simulink model "RADTRANS002"  (R2020b)
settings: Solver=VariableStepAuto  StartTime=0.0  StopTime=10.0  RelTol=1e-3
undefined symbols (not defined in the file): Line_110_C, Line_110_L, Line_110_R, Line_220_C, Line_220_L, Line_220_R, Line_35_C, Line_35_L, Line_35_R, Line_6_L, Line_6_R, Sys_f_Hz, Sys_V_net_kV, Tr_110_35_L_pu, Tr_110_35_R_pu, Tr_110_35_Sn_VA, Tr_110_35_V_HV_kV, Tr_110_35_V_LV_kV, Tr_110_6_L_pu, Tr_110_6_R_pu, Tr_110_6_Sn_VA, Tr_110_6_V_HV_kV, Tr_110_6_V_LV_kV, Tr_220_110_L_pu, Tr_220_110_R_pu, Tr_220_110_Sn_VA, Tr_220_110_V_HV_kV, Tr_220_110_V_LV_kV, Tr_35_04_L_pu, Tr_35_04_R_pu, Tr_35_04_Sn_VA, Tr_35_04_V_HV_kV, Tr_35_04_V_LV_kV, Tr_6_04_L_pu, Tr_6_04_R_pu, Tr_6_04_Sn_VA, Tr_6_04_V_HV_kV, Tr_6_04_V_LV_kV, Ts_powergui
libraries: dspstat3 x288, powerlib x202, powerlib_meascontrol x72
(part 1 of 7)
settings Model: Creator=New-life  LastModifiedBy=New-life

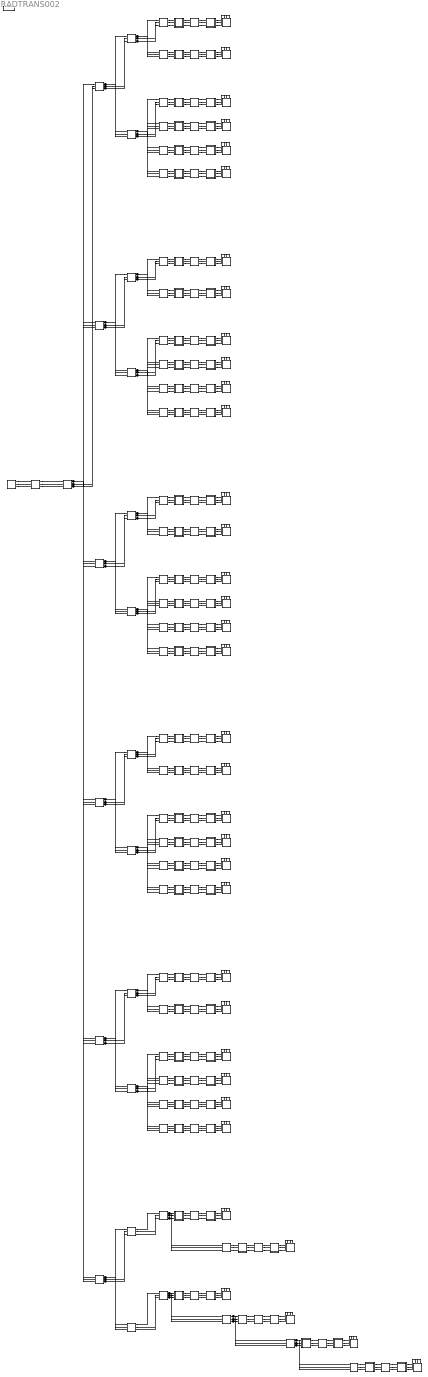
== system RADTRANS002 ==
  M_IN_Город_1_1 : Subsystem
      settings: CopyFcn=|
      | % Получаем путь и имя нового (только что скопированного) блока
      | blockPath = gcb;
      | blockName = get_param(blockPath, 'Name');
      | 
      | % Ищем число в названии самой подсистемы (например, берем "2" из "Measure_2")
      | numStr = regexp(blockName, '\d+', 'match');
      | 
      | if ~isempty(numStr)
      |     newNum = numStr{end}; % Берем последнее найденное число
      | 
      |     % --- 1. Обновляем скрытые теги в Goto и From (радиочастоты) ---
      |     gotos = find_system(blockPath, 'LookUnderMasks', 'on', 'BlockType', 'Goto');
      |     froms = find_system(blockPath, 'LookUnderMasks', 'on', 'BlockType', 'From');
      | 
      |     for i = 1:length(gotos)
      |         oldTag = get_param(gotos{i}, 'GotoTag');
      |         set_param(gotos{i}, 'GotoTag', regexprep(oldTag, '\d+$', newNum));
      |     end
      |     for i = 1:length(froms)
      |         oldTag = get_param(froms{i}, 'GotoTag');
      |         set_param(froms{i}, 'GotoTag', regexprep(oldTag, '\d+$', newNum));
      |     end
      | 
      |     % --- 2. ПЕРЕИМЕНОВЫВАЕМ САМИ БЛОКИ (визуальные надписи UI0 -> UI1 и т.д.) ---
      |     % Ищем все элементы только внутри этой подсистемы
      |     internalBlocks = find_system(blockPath, 'SearchDepth', 1, 'LookUnderMasks', 'on');
      | 
      |     % Цикл начинаем с 2, так как 1-й элемент в списке - это сама папка подсистемы
      |     for i = 2:length(internalBlocks)
      |         oldName = get_param(internalBlocks{i}, 'Name');
      |         % Ищем цифру в конце имени и меняем на новую
      |         newName = regexprep(oldName, '\d+$', newNum);
      | 
      |         % Если имя изменилось, применяем его
      |         if ~strcmp(oldName, newName)
      |             try
      |                 set_param(internalBlocks{i}, 'Name', newName);
      |             catch
      |                 % Игнорируем ошибку, если вдруг такое имя уже случайно есть
      |             end
      |         end
      |     end
      | end
  M_IN_Город_1_2 : Subsystem
      settings: CopyFcn=|
      | % Получаем путь и имя нового (только что скопированного) блока
      | blockPath = gcb;
      | blockName = get_param(blockPath, 'Name');
      | 
      | % Ищем число в названии самой подсистемы (например, берем "2" из "Measure_2")
      | numStr = regexp(blockName, '\d+', 'match');
      | 
      | if ~isempty(numStr)
      |     newNum = numStr{end}; % Берем последнее найденное число
      | 
      |     % --- 1. Обновляем скрытые теги в Goto и From (радиочастоты) ---
      |     gotos = find_system(blockPath, 'LookUnderMasks', 'on', 'BlockType', 'Goto');
      |     froms = find_system(blockPath, 'LookUnderMasks', 'on', 'BlockType', 'From');
      | 
      |     for i = 1:length(gotos)
      |         oldTag = get_param(gotos{i}, 'GotoTag');
      |         set_param(gotos{i}, 'GotoTag', regexprep(oldTag, '\d+$', newNum));
      |     end
      |     for i = 1:length(froms)
      |         oldTag = get_param(froms{i}, 'GotoTag');
      |         set_param(froms{i}, 'GotoTag', regexprep(oldTag, '\d+$', newNum));
      |     end
      | 
      |     % --- 2. ПЕРЕИМЕНОВЫВАЕМ САМИ БЛОКИ (визуальные надписи UI0 -> UI1 и т.д.) ---
      |     % Ищем все элементы только внутри этой подсистемы
      |     internalBlocks = find_system(blockPath, 'SearchDepth', 1, 'LookUnderMasks', 'on');
      | 
      |     % Цикл начинаем с 2, так как 1-й элемент в списке - это сама папка подсистемы
      |     for i = 2:length(internalBlocks)
      |         oldName = get_param(internalBlocks{i}, 'Name');
      |         % Ищем цифру в конце имени и меняем на новую
      |         newName = regexprep(oldName, '\d+$', newNum);
      | 
      |         % Если имя изменилось, применяем его
      |         if ~strcmp(oldName, newName)
      |             try
      |                 set_param(internalBlocks{i}, 'Name', newName);
      |             catch
      |                 % Игнорируем ошибку, если вдруг такое имя уже случайно есть
      |             end
      |         end
      |     end
      | end
  M_IN_Город_1_3 : Subsystem
      settings: CopyFcn=|
      | % Получаем путь и имя нового (только что скопированного) блока
      | blockPath = gcb;
      | blockName = get_param(blockPath, 'Name');
      | 
      | % Ищем число в названии самой подсистемы (например, берем "2" из "Measure_2")
      | numStr = regexp(blockName, '\d+', 'match');
      | 
      | if ~isempty(numStr)
      |     newNum = numStr{end}; % Берем последнее найденное число
      | 
      |     % --- 1. Обновляем скрытые теги в Goto и From (радиочастоты) ---
      |     gotos = find_system(blockPath, 'LookUnderMasks', 'on', 'BlockType', 'Goto');
      |     froms = find_system(blockPath, 'LookUnderMasks', 'on', 'BlockType', 'From');
      | 
      |     for i = 1:length(gotos)
      |         oldTag = get_param(gotos{i}, 'GotoTag');
      |         set_param(gotos{i}, 'GotoTag', regexprep(oldTag, '\d+$', newNum));
      |     end
      |     for i = 1:length(froms)
      |         oldTag = get_param(froms{i}, 'GotoTag');
      |         set_param(froms{i}, 'GotoTag', regexprep(oldTag, '\d+$', newNum));
      |     end
      | 
      |     % --- 2. ПЕРЕИМЕНОВЫВАЕМ САМИ БЛОКИ (визуальные надписи UI0 -> UI1 и т.д.) ---
      |     % Ищем все элементы только внутри этой подсистемы
      |     internalBlocks = find_system(blockPath, 'SearchDepth', 1, 'LookUnderMasks', 'on');
      | 
      |     % Цикл начинаем с 2, так как 1-й элемент в списке - это сама папка подсистемы
      |     for i = 2:length(internalBlocks)
      |         oldName = get_param(internalBlocks{i}, 'Name');
      |         % Ищем цифру в конце имени и меняем на новую
      |         newName = regexprep(oldName, '\d+$', newNum);
      | 
      |         % Если имя изменилось, применяем его
      |         if ~strcmp(oldName, newName)
      |             try
      |                 set_param(internalBlocks{i}, 'Name', newName);
      |             catch
      |                 % Игнорируем ошибку, если вдруг такое имя уже случайно есть
      |             end
      |         end
      |     end
      | end
  M_IN_Город_1_4 : Subsystem
      settings: CopyFcn=|
      | % Получаем путь и имя нового (только что скопированного) блока
      | blockPath = gcb;
      | blockName = get_param(blockPath, 'Name');
      | 
      | % Ищем число в названии самой подсистемы (например, берем "2" из "Measure_2")
      | numStr = regexp(blockName, '\d+', 'match');
      | 
      | if ~isempty(numStr)
      |     newNum = numStr{end}; % Берем последнее найденное число
      | 
      |     % --- 1. Обновляем скрытые теги в Goto и From (радиочастоты) ---
      |     gotos = find_system(blockPath, 'LookUnderMasks', 'on', 'BlockType', 'Goto');
      |     froms = find_system(blockPath, 'LookUnderMasks', 'on', 'BlockType', 'From');
      | 
      |     for i = 1:length(gotos)
      |         oldTag = get_param(gotos{i}, 'GotoTag');
      |         set_param(gotos{i}, 'GotoTag', regexprep(oldTag, '\d+$', newNum));
      |     end
      |     for i = 1:length(froms)
      |         oldTag = get_param(froms{i}, 'GotoTag');
      |         set_param(froms{i}, 'GotoTag', regexprep(oldTag, '\d+$', newNum));
      |     end
      | 
      |     % --- 2. ПЕРЕИМЕНОВЫВАЕМ САМИ БЛОКИ (визуальные надписи UI0 -> UI1 и т.д.) ---
      |     % Ищем все элементы только внутри этой подсистемы
      |     internalBlocks = find_system(blockPath, 'SearchDepth', 1, 'LookUnderMasks', 'on');
      | 
      |     % Цикл начинаем с 2, так как 1-й элемент в списке - это сама папка подсистемы
      |     for i = 2:length(internalBlocks)
      |         oldName = get_param(internalBlocks{i}, 'Name');
      |         % Ищем цифру в конце имени и меняем на новую
      |         newName = regexprep(oldName, '\d+$', newNum);
      | 
      |         % Если имя изменилось, применяем его
      |         if ~strcmp(oldName, newName)
      |             try
      |                 set_param(internalBlocks{i}, 'Name', newName);
      |             catch
      |                 % Игнорируем ошибку, если вдруг такое имя уже случайно есть
      |             end
      |         end
      |     end
      | end
  M_IN_Город_2_1 : Subsystem
      settings: CopyFcn=|
      | % Получаем путь и имя нового (только что скопированного) блока
      | blockPath = gcb;
      | blockName = get_param(blockPath, 'Name');
      | 
      | % Ищем число в названии самой подсистемы (например, берем "2" из "Measure_2")
      | numStr = regexp(blockName, '\d+', 'match');
      | 
      | if ~isempty(numStr)
      |     newNum = numStr{end}; % Берем последнее найденное число
      | 
      |     % --- 1. Обновляем скрытые теги в Goto и From (радиочастоты) ---
      |     gotos = find_system(blockPath, 'LookUnderMasks', 'on', 'BlockType', 'Goto');
      |     froms = find_system(blockPath, 'LookUnderMasks', 'on', 'BlockType', 'From');
      | 
      |     for i = 1:length(gotos)
      |         oldTag = get_param(gotos{i}, 'GotoTag');
      |         set_param(gotos{i}, 'GotoTag', regexprep(oldTag, '\d+$', newNum));
      |     end
      |     for i = 1:length(froms)
      |         oldTag = get_param(froms{i}, 'GotoTag');
      |         set_param(froms{i}, 'GotoTag', regexprep(oldTag, '\d+$', newNum));
      |     end
      | 
      |     % --- 2. ПЕРЕИМЕНОВЫВАЕМ САМИ БЛОКИ (визуальные надписи UI0 -> UI1 и т.д.) ---
      |     % Ищем все элементы только внутри этой подсистемы
      |     internalBlocks = find_system(blockPath, 'SearchDepth', 1, 'LookUnderMasks', 'on');
      | 
      |     % Цикл начинаем с 2, так как 1-й элемент в списке - это сама папка подсистемы
      |     for i = 2:length(internalBlocks)
      |         oldName = get_param(internalBlocks{i}, 'Name');
      |         % Ищем цифру в конце имени и меняем на новую
      |         newName = regexprep(oldName, '\d+$', newNum);
      | 
      |         % Если имя изменилось, применяем его
      |         if ~strcmp(oldName, newName)
      |             try
      |                 set_param(internalBlocks{i}, 'Name', newName);
      |             catch
      |                 % Игнорируем ошибку, если вдруг такое имя уже случайно есть
      |             end
      |         end
      |     end
      | end
  M_IN_Город_2_2 : Subsystem
      settings: CopyFcn=|
      | % Получаем путь и имя нового (только что скопированного) блока
      | blockPath = gcb;
      | blockName = get_param(blockPath, 'Name');
      | 
      | % Ищем число в названии самой подсистемы (например, берем "2" из "Measure_2")
      | numStr = regexp(blockName, '\d+', 'match');
      | 
      | if ~isempty(numStr)
      |     newNum = numStr{end}; % Берем последнее найденное число
      | 
      |     % --- 1. Обновляем скрытые теги в Goto и From (радиочастоты) ---
      |     gotos = find_system(blockPath, 'LookUnderMasks', 'on', 'BlockType', 'Goto');
      |     froms = find_system(blockPath, 'LookUnderMasks', 'on', 'BlockType', 'From');
      | 
      |     for i = 1:length(gotos)
      |         oldTag = get_param(gotos{i}, 'GotoTag');
      |         set_param(gotos{i}, 'GotoTag', regexprep(oldTag, '\d+$', newNum));
      |     end
      |     for i = 1:length(froms)
      |         oldTag = get_param(froms{i}, 'GotoTag');
      |         set_param(froms{i}, 'GotoTag', regexprep(oldTag, '\d+$', newNum));
      |     end
      | 
      |     % --- 2. ПЕРЕИМЕНОВЫВАЕМ САМИ БЛОКИ (визуальные надписи UI0 -> UI1 и т.д.) ---
      |     % Ищем все элементы только внутри этой подсистемы
      |     internalBlocks = find_system(blockPath, 'SearchDepth', 1, 'LookUnderMasks', 'on');
      | 
      |     % Цикл начинаем с 2, так как 1-й элемент в списке - это сама папка подсистемы
      |     for i = 2:length(internalBlocks)
      |         oldName = get_param(internalBlocks{i}, 'Name');
      |         % Ищем цифру в конце имени и меняем на новую
      |         newName = regexprep(oldName, '\d+$', newNum);
      | 
      |         % Если имя изменилось, применяем его
      |         if ~strcmp(oldName, newName)
      |             try
      |                 set_param(internalBlocks{i}, 'Name', newName);
      |             catch
      |                 % Игнорируем ошибку, если вдруг такое имя уже случайно есть
      |             end
      |         end
      |     end
      | end
  M_IN_Город_2_3 : Subsystem
      settings: CopyFcn=|
      | % Получаем путь и имя нового (только что скопированного) блока
      | blockPath = gcb;
      | blockName = get_param(blockPath, 'Name');
      | 
      | % Ищем число в названии самой подсистемы (например, берем "2" из "Measure_2")
      | numStr = regexp(blockName, '\d+', 'match');
      | 
      | if ~isempty(numStr)
      |     newNum = numStr{end}; % Берем последнее найденное число
      | 
      |     % --- 1. Обновляем скрытые теги в Goto и From (радиочастоты) ---
      |     gotos = find_system(blockPath, 'LookUnderMasks', 'on', 'BlockType', 'Goto');
      |     froms = find_system(blockPath, 'LookUnderMasks', 'on', 'BlockType', 'From');
      | 
      |     for i = 1:length(gotos)
      |         oldTag = get_param(gotos{i}, 'GotoTag');
      |         set_param(gotos{i}, 'GotoTag', regexprep(oldTag, '\d+$', newNum));
      |     end
      |     for i = 1:length(froms)
      |         oldTag = get_param(froms{i}, 'GotoTag');
      |         set_param(froms{i}, 'GotoTag', regexprep(oldTag, '\d+$', newNum));
      |     end
      | 
      |     % --- 2. ПЕРЕИМЕНОВЫВАЕМ САМИ БЛОКИ (визуальные надписи UI0 -> UI1 и т.д.) ---
      |     % Ищем все элементы только внутри этой подсистемы
      |     internalBlocks = find_system(blockPath, 'SearchDepth', 1, 'LookUnderMasks', 'on');
      | 
      |     % Цикл начинаем с 2, так как 1-й элемент в списке - это сама папка подсистемы
      |     for i = 2:length(internalBlocks)
      |         oldName = get_param(internalBlocks{i}, 'Name');
      |         % Ищем цифру в конце имени и меняем на новую
      |         newName = regexprep(oldName, '\d+$', newNum);
      | 
      |         % Если имя изменилось, применяем его
      |         if ~strcmp(oldName, newName)
      |             try
      |                 set_param(internalBlocks{i}, 'Name', newName);
      |             catch
      |                 % Игнорируем ошибку, если вдруг такое имя уже случайно есть
      |             end
      |         end
      |     end
      | end
  M_IN_Город_2_4 : Subsystem
      settings: CopyFcn=|
      | % Получаем путь и имя нового (только что скопированного) блока
      | blockPath = gcb;
      | blockName = get_param(blockPath, 'Name');
      | 
      | % Ищем число в названии самой подсистемы (например, берем "2" из "Measure_2")
      | numStr = regexp(blockName, '\d+', 'match');
      | 
      | if ~isempty(numStr)
      |     newNum = numStr{end}; % Берем последнее найденное число
      | 
      |     % --- 1. Обновляем скрытые теги в Goto и From (радиочастоты) ---
      |     gotos = find_system(blockPath, 'LookUnderMasks', 'on', 'BlockType', 'Goto');
      |     froms = find_system(blockPath, 'LookUnderMasks', 'on', 'BlockType', 'From');
      | 
      |     for i = 1:length(gotos)
      |         oldTag = get_param(gotos{i}, 'GotoTag');
      |         set_param(gotos{i}, 'GotoTag', regexprep(oldTag, '\d+$', newNum));
      |     end
      |     for i = 1:length(froms)
      |         oldTag = get_param(froms{i}, 'GotoTag');
      |         set_param(froms{i}, 'GotoTag', regexprep(oldTag, '\d+$', newNum));
      |     end
      | 
      |     % --- 2. ПЕРЕИМЕНОВЫВАЕМ САМИ БЛОКИ (визуальные надписи UI0 -> UI1 и т.д.) ---
      |     % Ищем все элементы только внутри этой подсистемы
      |     internalBlocks = find_system(blockPath, 'SearchDepth', 1, 'LookUnderMasks', 'on');
      | 
      |     % Цикл начинаем с 2, так как 1-й элемент в списке - это сама папка подсистемы
      |     for i = 2:length(internalBlocks)
      |         oldName = get_param(internalBlocks{i}, 'Name');
      |         % Ищем цифру в конце имени и меняем на новую
      |         newName = regexprep(oldName, '\d+$', newNum);
      | 
      |         % Если имя изменилось, применяем его
      |         if ~strcmp(oldName, newName)
      |             try
      |                 set_param(internalBlocks{i}, 'Name', newName);
      |             catch
      |                 % Игнорируем ошибку, если вдруг такое имя уже случайно есть
      |             end
      |         end
      |     end
      | end
  M_IN_Город_3_1 : Subsystem
      settings: CopyFcn=|
      | % Получаем путь и имя нового (только что скопированного) блока
      | blockPath = gcb;
      | blockName = get_param(blockPath, 'Name');
      | 
      | % Ищем число в названии самой подсистемы (например, берем "2" из "Measure_2")
      | numStr = regexp(blockName, '\d+', 'match');
      | 
      | if ~isempty(numStr)
      |     newNum = numStr{end}; % Берем последнее найденное число
      | 
      |     % --- 1. Обновляем скрытые теги в Goto и From (радиочастоты) ---
      |     gotos = find_system(blockPath, 'LookUnderMasks', 'on', 'BlockType', 'Goto');
      |     froms = find_system(blockPath, 'LookUnderMasks', 'on', 'BlockType', 'From');
      | 
      |     for i = 1:length(gotos)
      |         oldTag = get_param(gotos{i}, 'GotoTag');
      |         set_param(gotos{i}, 'GotoTag', regexprep(oldTag, '\d+$', newNum));
      |     end
      |     for i = 1:length(froms)
      |         oldTag = get_param(froms{i}, 'GotoTag');
      |         set_param(froms{i}, 'GotoTag', regexprep(oldTag, '\d+$', newNum));
      |     end
      | 
      |     % --- 2. ПЕРЕИМЕНОВЫВАЕМ САМИ БЛОКИ (визуальные надписи UI0 -> UI1 и т.д.) ---
      |     % Ищем все элементы только внутри этой подсистемы
      |     internalBlocks = find_system(blockPath, 'SearchDepth', 1, 'LookUnderMasks', 'on');
      | 
      |     % Цикл начинаем с 2, так как 1-й элемент в списке - это сама папка подсистемы
      |     for i = 2:length(internalBlocks)
      |         oldName = get_param(internalBlocks{i}, 'Name');
      |         % Ищем цифру в конце имени и меняем на новую
      |         newName = regexprep(oldName, '\d+$', newNum);
      | 
      |         % Если имя изменилось, применяем его
      |         if ~strcmp(oldName, newName)
      |             try
      |                 set_param(internalBlocks{i}, 'Name', newName);
      |             catch
      |                 % Игнорируем ошибку, если вдруг такое имя уже случайно есть
      |             end
      |         end
      |     end
      | end
  M_IN_Город_3_2 : Subsystem
      settings: CopyFcn=|
      | % Получаем путь и имя нового (только что скопированного) блока
      | blockPath = gcb;
      | blockName = get_param(blockPath, 'Name');
      | 
      | % Ищем число в названии самой подсистемы (например, берем "2" из "Measure_2")
      | numStr = regexp(blockName, '\d+', 'match');
      | 
      | if ~isempty(numStr)
      |     newNum = numStr{end}; % Берем последнее найденное число
      | 
      |     % --- 1. Обновляем скрытые теги в Goto и From (радиочастоты) ---
      |     gotos = find_system(blockPath, 'LookUnderMasks', 'on', 'BlockType', 'Goto');
      |     froms = find_system(blockPath, 'LookUnderMasks', 'on', 'BlockType', 'From');
      | 
      |     for i = 1:length(gotos)
      |         oldTag = get_param(gotos{i}, 'GotoTag');
      |         set_param(gotos{i}, 'GotoTag', regexprep(oldTag, '\d+$', newNum));
      |     end
      |     for i = 1:length(froms)
      |         oldTag = get_param(froms{i}, 'GotoTag');
      |         set_param(froms{i}, 'GotoTag', regexprep(oldTag, '\d+$', newNum));
      |     end
      | 
      |     % --- 2. ПЕРЕИМЕНОВЫВАЕМ САМИ БЛОКИ (визуальные надписи UI0 -> UI1 и т.д.) ---
      |     % Ищем все элементы только внутри этой подсистемы
      |     internalBlocks = find_system(blockPath, 'SearchDepth', 1, 'LookUnderMasks', 'on');
      | 
      |     % Цикл начинаем с 2, так как 1-й элемент в списке - это сама папка подсистемы
      |     for i = 2:length(internalBlocks)
      |         oldName = get_param(internalBlocks{i}, 'Name');
      |         % Ищем цифру в конце имени и меняем на новую
      |         newName = regexprep(oldName, '\d+$', newNum);
      | 
      |         % Если имя изменилось, применяем его
      |         if ~strcmp(oldName, newName)
      |             try
      |                 set_param(internalBlocks{i}, 'Name', newName);
      |             catch
      |                 % Игнорируем ошибку, если вдруг такое имя уже случайно есть
      |             end
      |         end
      |     end
      | end
  M_IN_Город_3_3 : Subsystem
      settings: CopyFcn=|
      | % Получаем путь и имя нового (только что скопированного) блока
      | blockPath = gcb;
      | blockName = get_param(blockPath, 'Name');
      | 
      | % Ищем число в названии самой подсистемы (например, берем "2" из "Measure_2")
      | numStr = regexp(blockName, '\d+', 'match');
      | 
      | if ~isempty(numStr)
      |     newNum = numStr{end}; % Берем последнее найденное число
      | 
      |     % --- 1. Обновляем скрытые теги в Goto и From (радиочастоты) ---
      |     gotos = find_system(blockPath, 'LookUnderMasks', 'on', 'BlockType', 'Goto');
      |     froms = find_system(blockPath, 'LookUnderMasks', 'on', 'BlockType', 'From');
      | 
      |     for i = 1:length(gotos)
      |         oldTag = get_param(gotos{i}, 'GotoTag');
      |         set_param(gotos{i}, 'GotoTag', regexprep(oldTag, '\d+$', newNum));
      |     end
      |     for i = 1:length(froms)
      |         oldTag = get_param(froms{i}, 'GotoTag');
      |         set_param(froms{i}, 'GotoTag', regexprep(oldTag, '\d+$', newNum));
      |     end
      | 
      |     % --- 2. ПЕРЕИМЕНОВЫВАЕМ САМИ БЛОКИ (визуальные надписи UI0 -> UI1 и т.д.) ---
      |     % Ищем все элементы только внутри этой подсистемы
      |     internalBlocks = find_system(blockPath, 'SearchDepth', 1, 'LookUnderMasks', 'on');
      | 
      |     % Цикл начинаем с 2, так как 1-й элемент в списке - это сама папка подсистемы
      |     for i = 2:length(internalBlocks)
      |         oldName = get_param(internalBlocks{i}, 'Name');
      |         % Ищем цифру в конце имени и меняем на новую
      |         newName = regexprep(oldName, '\d+$', newNum);
      | 
      |         % Если имя изменилось, применяем его
      |         if ~strcmp(oldName, newName)
      |             try
      |                 set_param(internalBlocks{i}, 'Name', newName);
      |             catch
      |                 % Игнорируем ошибку, если вдруг такое имя уже случайно есть
      |             end
      |         end
      |     end
      | end
  M_IN_Город_3_4 : Subsystem
      settings: CopyFcn=|
      | % Получаем путь и имя нового (только что скопированного) блока
      | blockPath = gcb;
      | blockName = get_param(blockPath, 'Name');
      | 
      | % Ищем число в названии самой подсистемы (например, берем "2" из "Measure_2")
      | numStr = regexp(blockName, '\d+', 'match');
      | 
      | if ~isempty(numStr)
      |     newNum = numStr{end}; % Берем последнее найденное число
      | 
      |     % --- 1. Обновляем скрытые теги в Goto и From (радиочастоты) ---
      |     gotos = find_system(blockPath, 'LookUnderMasks', 'on', 'BlockType', 'Goto');
      |     froms = find_system(blockPath, 'LookUnderMasks', 'on', 'BlockType', 'From');
      | 
      |     for i = 1:length(gotos)
      |         oldTag = get_param(gotos{i}, 'GotoTag');
      |         set_param(gotos{i}, 'GotoTag', regexprep(oldTag, '\d+$', newNum));
      |     end
      |     for i = 1:length(froms)
      |         oldTag = get_param(froms{i}, 'GotoTag');
      |         set_param(froms{i}, 'GotoTag', regexprep(oldTag, '\d+$', newNum));
      |     end
      | 
      |     % --- 2. ПЕРЕИМЕНОВЫВАЕМ САМИ БЛОКИ (визуальные надписи UI0 -> UI1 и т.д.) ---
      |     % Ищем все элементы только внутри этой подсистемы
      |     internalBlocks = find_system(blockPath, 'SearchDepth', 1, 'LookUnderMasks', 'on');
      | 
      |     % Цикл начинаем с 2, так как 1-й элемент в списке - это сама папка подсистемы
      |     for i = 2:length(internalBlocks)
      |         oldName = get_param(internalBlocks{i}, 'Name');
      |         % Ищем цифру в конце имени и меняем на новую
      |         newName = regexprep(oldName, '\d+$', newNum);
      | 
      |         % Если имя изменилось, применяем его
      |         if ~strcmp(oldName, newName)
      |             try
      |                 set_param(internalBlocks{i}, 'Name', newName);
      |             catch
      |                 % Игнорируем ошибку, если вдруг такое имя уже случайно есть
      |             end
      |         end
      |     end
      | end
  M_IN_Город_4_1 : Subsystem
      settings: CopyFcn=|
      | % Получаем путь и имя нового (только что скопированного) блока
      | blockPath = gcb;
      | blockName = get_param(blockPath, 'Name');
      | 
      | % Ищем число в названии самой подсистемы (например, берем "2" из "Measure_2")
      | numStr = regexp(blockName, '\d+', 'match');
      | 
      | if ~isempty(numStr)
      |     newNum = numStr{end}; % Берем последнее найденное число
      | 
      |     % --- 1. Обновляем скрытые теги в Goto и From (радиочастоты) ---
      |     gotos = find_system(blockPath, 'LookUnderMasks', 'on', 'BlockType', 'Goto');
      |     froms = find_system(blockPath, 'LookUnderMasks', 'on', 'BlockType', 'From');
      | 
      |     for i = 1:length(gotos)
      |         oldTag = get_param(gotos{i}, 'GotoTag');
      |         set_param(gotos{i}, 'GotoTag', regexprep(oldTag, '\d+$', newNum));
      |     end
      |     for i = 1:length(froms)
      |         oldTag = get_param(froms{i}, 'GotoTag');
      |         set_param(froms{i}, 'GotoTag', regexprep(oldTag, '\d+$', newNum));
      |     end
      | 
      |     % --- 2. ПЕРЕИМЕНОВЫВАЕМ САМИ БЛОКИ (визуальные надписи UI0 -> UI1 и т.д.) ---
      |     % Ищем все элементы только внутри этой подсистемы
      |     internalBlocks = find_system(blockPath, 'SearchDepth', 1, 'LookUnderMasks', 'on');
      | 
      |     % Цикл начинаем с 2, так как 1-й элемент в списке - это сама папка подсистемы
      |     for i = 2:length(internalBlocks)
      |         oldName = get_param(internalBlocks{i}, 'Name');
      |         % Ищем цифру в конце имени и меняем на новую
      |         newName = regexprep(oldName, '\d+$', newNum);
      | 
      |         % Если имя изменилось, применяем его
      |         if ~strcmp(oldName, newName)
      |             try
      |                 set_param(internalBlocks{i}, 'Name', newName);
      |             catch
      |                 % Игнорируем ошибку, если вдруг такое имя уже случайно есть
      |             end
      |         end
      |     end
      | end
  M_IN_Город_4_2 : Subsystem
      settings: CopyFcn=|
      | % Получаем путь и имя нового (только что скопированного) блока
      | blockPath = gcb;
      | blockName = get_param(blockPath, 'Name');
      | 
      | % Ищем число в названии самой подсистемы (например, берем "2" из "Measure_2")
      | numStr = regexp(blockName, '\d+', 'match');
      | 
      | if ~isempty(numStr)
      |     newNum = numStr{end}; % Берем последнее найденное число
      | 
      |     % --- 1. Обновляем скрытые теги в Goto и From (радиочастоты) ---
      |     gotos = find_system(blockPath, 'LookUnderMasks', 'on', 'BlockType', 'Goto');
      |     froms = find_system(blockPath, 'LookUnderMasks', 'on', 'BlockType', 'From');
      | 
      |     for i = 1:length(gotos)
      |         oldTag = get_param(gotos{i}, 'GotoTag');
      |         set_param(gotos{i}, 'GotoTag', regexprep(oldTag, '\d+$', newNum));
      |     end
      |     for i = 1:length(froms)
      |         oldTag = get_param(froms{i}, 'GotoTag');
      |         set_param(froms{i}, 'GotoTag', regexprep(oldTag, '\d+$', newNum));
      |     end
      | 
      |     % --- 2. ПЕРЕИМЕНОВЫВАЕМ САМИ БЛОКИ (визуальные надписи UI0 -> UI1 и т.д.) ---
      |     % Ищем все элементы только внутри этой подсистемы
      |     internalBlocks = find_system(blockPath, 'SearchDepth', 1, 'LookUnderMasks', 'on');
      | 
      |     % Цикл начинаем с 2, так как 1-й элемент в списке - это сама папка подсистемы
      |     for i = 2:length(internalBlocks)
      |         oldName = get_param(internalBlocks{i}, 'Name');
      |         % Ищем цифру в конце имени и меняем на новую
      |         newName = regexprep(oldName, '\d+$', newNum);
      | 
      |         % Если имя изменилось, применяем его
      |         if ~strcmp(oldName, newName)
      |             try
      |                 set_param(internalBlocks{i}, 'Name', newName);
      |             catch
      |                 % Игнорируем ошибку, если вдруг такое имя уже случайно есть
      |             end
      |         end
      |     end
      | end
  M_IN_Город_4_3 : Subsystem
      settings: CopyFcn=|
      | % Получаем путь и имя нового (только что скопированного) блока
      | blockPath = gcb;
      | blockName = get_param(blockPath, 'Name');
      | 
      | % Ищем число в названии самой подсистемы (например, берем "2" из "Measure_2")
      | numStr = regexp(blockName, '\d+', 'match');
      | 
      | if ~isempty(numStr)
      |     newNum = numStr{end}; % Берем последнее найденное число
      | 
      |     % --- 1. Обновляем скрытые теги в Goto и From (радиочастоты) ---
      |     gotos = find_system(blockPath, 'LookUnderMasks', 'on', 'BlockType', 'Goto');
      |     froms = find_system(blockPath, 'LookUnderMasks', 'on', 'BlockType', 'From');
      | 
      |     for i = 1:length(gotos)
      |         oldTag = get_param(gotos{i}, 'GotoTag');
      |         set_param(gotos{i}, 'GotoTag', regexprep(oldTag, '\d+$', newNum));
      |     end
      |     for i = 1:length(froms)
      |         oldTag = get_param(froms{i}, 'GotoTag');
      |         set_param(froms{i}, 'GotoTag', regexprep(oldTag, '\d+$', newNum));
      |     end
      | 
      |     % --- 2. ПЕРЕИМЕНОВЫВАЕМ САМИ БЛОКИ (визуальные надписи UI0 -> UI1 и т.д.) ---
      |     % Ищем все элементы только внутри этой подсистемы
      |     internalBlocks = find_system(blockPath, 'SearchDepth', 1, 'LookUnderMasks', 'on');
      | 
      |     % Цикл начинаем с 2, так как 1-й элемент в списке - это сама папка подсистемы
      |     for i = 2:length(internalBlocks)
      |         oldName = get_param(internalBlocks{i}, 'Name');
      |         % Ищем цифру в конце имени и меняем на новую
      |         newName = regexprep(oldName, '\d+$', newNum);
      | 
      |         % Если имя изменилось, применяем его
      |         if ~strcmp(oldName, newName)
      |             try
      |                 set_param(internalBlocks{i}, 'Name', newName);
      |             catch
      |                 % Игнорируем ошибку, если вдруг такое имя уже случайно есть
      |             end
      |         end
      |     end
      | end
  M_IN_Город_4_4 : Subsystem
      settings: CopyFcn=|
      | % Получаем путь и имя нового (только что скопированного) блока
      | blockPath = gcb;
      | blockName = get_param(blockPath, 'Name');
      | 
      | % Ищем число в названии самой подсистемы (например, берем "2" из "Measure_2")
      | numStr = regexp(blockName, '\d+', 'match');
      | 
      | if ~isempty(numStr)
      |     newNum = numStr{end}; % Берем последнее найденное число
      | 
      |     % --- 1. Обновляем скрытые теги в Goto и From (радиочастоты) ---
      |     gotos = find_system(blockPath, 'LookUnderMasks', 'on', 'BlockType', 'Goto');
      |     froms = find_system(blockPath, 'LookUnderMasks', 'on', 'BlockType', 'From');
      | 
      |     for i = 1:length(gotos)
      |         oldTag = get_param(gotos{i}, 'GotoTag');
      |         set_param(gotos{i}, 'GotoTag', regexprep(oldTag, '\d+$', newNum));
      |     end
      |     for i = 1:length(froms)
      |         oldTag = get_param(froms{i}, 'GotoTag');
      |         set_param(froms{i}, 'GotoTag', regexprep(oldTag, '\d+$', newNum));
      |     end
      | 
      |     % --- 2. ПЕРЕИМЕНОВЫВАЕМ САМИ БЛОКИ (визуальные надписи UI0 -> UI1 и т.д.) ---
      |     % Ищем все элементы только внутри этой подсистемы
      |     internalBlocks = find_system(blockPath, 'SearchDepth', 1, 'LookUnderMasks', 'on');
      | 
      |     % Цикл начинаем с 2, так как 1-й элемент в списке - это сама папка подсистемы
      |     for i = 2:length(internalBlocks)
      |         oldName = get_param(internalBlocks{i}, 'Name');
      |         % Ищем цифру в конце имени и меняем на новую
      |         newName = regexprep(oldName, '\d+$', newNum);
      | 
      |         % Если имя изменилось, применяем его
      |         if ~strcmp(oldName, newName)
      |             try
      |                 set_param(internalBlocks{i}, 'Name', newName);
      |             catch
      |                 % Игнорируем ошибку, если вдруг такое имя уже случайно есть
      |             end
      |         end
      |     end
      | end
  M_IN_Город_5_1 : Subsystem
      settings: CopyFcn=|
      | % Получаем путь и имя нового (только что скопированного) блока
      | blockPath = gcb;
      | blockName = get_param(blockPath, 'Name');
      | 
      | % Ищем число в названии самой подсистемы (например, берем "2" из "Measure_2")
      | numStr = regexp(blockName, '\d+', 'match');
      | 
      | if ~isempty(numStr)
      |     newNum = numStr{end}; % Берем последнее найденное число
      | 
      |     % --- 1. Обновляем скрытые теги в Goto и From (радиочастоты) ---
      |     gotos = find_system(blockPath, 'LookUnderMasks', 'on', 'BlockType', 'Goto');
      |     froms = find_system(blockPath, 'LookUnderMasks', 'on', 'BlockType', 'From');
      | 
      |     for i = 1:length(gotos)
      |         oldTag = get_param(gotos{i}, 'GotoTag');
      |         set_param(gotos{i}, 'GotoTag', regexprep(oldTag, '\d+$', newNum));
      |     end
      |     for i = 1:length(froms)
      |         oldTag = get_param(froms{i}, 'GotoTag');
      |         set_param(froms{i}, 'GotoTag', regexprep(oldTag, '\d+$', newNum));
      |     end
      | 
      |     % --- 2. ПЕРЕИМЕНОВЫВАЕМ САМИ БЛОКИ (визуальные надписи UI0 -> UI1 и т.д.) ---
      |     % Ищем все элементы только внутри этой подсистемы
      |     internalBlocks = find_system(blockPath, 'SearchDepth', 1, 'LookUnderMasks', 'on');
      | 
      |     % Цикл начинаем с 2, так как 1-й элемент в списке - это сама папка подсистемы
      |     for i = 2:length(internalBlocks)
      |         oldName = get_param(internalBlocks{i}, 'Name');
      |         % Ищем цифру в конце имени и меняем на новую
      |         newName = regexprep(oldName, '\d+$', newNum);
      | 
      |         % Если имя изменилось, применяем его
      |         if ~strcmp(oldName, newName)
      |             try
      |                 set_param(internalBlocks{i}, 'Name', newName);
      |             catch
      |                 % Игнорируем ошибку, если вдруг такое имя уже случайно есть
      |             end
      |         end
      |     end
      | end
  M_IN_Город_5_2 : Subsystem
      settings: CopyFcn=|
      | % Получаем путь и имя нового (только что скопированного) блока
      | blockPath = gcb;
      | blockName = get_param(blockPath, 'Name');
      | 
      | % Ищем число в названии самой подсистемы (например, берем "2" из "Measure_2")
      | numStr = regexp(blockName, '\d+', 'match');
      | 
      | if ~isempty(numStr)
      |     newNum = numStr{end}; % Берем последнее найденное число
      | 
      |     % --- 1. Обновляем скрытые теги в Goto и From (радиочастоты) ---
      |     gotos = find_system(blockPath, 'LookUnderMasks', 'on', 'BlockType', 'Goto');
      |     froms = find_system(blockPath, 'LookUnderMasks', 'on', 'BlockType', 'From');
      | 
      |     for i = 1:length(gotos)
      |         oldTag = get_param(gotos{i}, 'GotoTag');
      |         set_param(gotos{i}, 'GotoTag', regexprep(oldTag, '\d+$', newNum));
      |     end
      |     for i = 1:length(froms)
      |         oldTag = get_param(froms{i}, 'GotoTag');
      |         set_param(froms{i}, 'GotoTag', regexprep(oldTag, '\d+$', newNum));
      |     end
      | 
      |     % --- 2. ПЕРЕИМЕНОВЫВАЕМ САМИ БЛОКИ (визуальные надписи UI0 -> UI1 и т.д.) ---
      |     % Ищем все элементы только внутри этой подсистемы
      |     internalBlocks = find_system(blockPath, 'SearchDepth', 1, 'LookUnderMasks', 'on');
      | 
      |     % Цикл начинаем с 2, так как 1-й элемент в списке - это сама папка подсистемы
      |     for i = 2:length(internalBlocks)
      |         oldName = get_param(internalBlocks{i}, 'Name');
      |         % Ищем цифру в конце имени и меняем на новую
      |         newName = regexprep(oldName, '\d+$', newNum);
      | 
      |         % Если имя изменилось, применяем его
      |         if ~strcmp(oldName, newName)
      |             try
      |                 set_param(internalBlocks{i}, 'Name', newName);
      |             catch
      |                 % Игнорируем ошибку, если вдруг такое имя уже случайно есть
      |             end
      |         end
      |     end
      | end
  M_IN_Город_5_3 : Subsystem
      settings: CopyFcn=|
      | % Получаем путь и имя нового (только что скопированного) блока
      | blockPath = gcb;
      | blockName = get_param(blockPath, 'Name');
      | 
      | % Ищем число в названии самой подсистемы (например, берем "2" из "Measure_2")
      | numStr = regexp(blockName, '\d+', 'match');
      | 
      | if ~isempty(numStr)
      |     newNum = numStr{end}; % Берем последнее найденное число
      | 
      |     % --- 1. Обновляем скрытые теги в Goto и From (радиочастоты) ---
      |     gotos = find_system(blockPath, 'LookUnderMasks', 'on', 'BlockType', 'Goto');
      |     froms = find_system(blockPath, 'LookUnderMasks', 'on', 'BlockType', 'From');
      | 
      |     for i = 1:length(gotos)
      |         oldTag = get_param(gotos{i}, 'GotoTag');
      |         set_param(gotos{i}, 'GotoTag', regexprep(oldTag, '\d+$', newNum));
      |     end
      |     for i = 1:length(froms)
      |         oldTag = get_param(froms{i}, 'GotoTag');
      |         set_param(froms{i}, 'GotoTag', regexprep(oldTag, '\d+$', newNum));
      |     end
      | 
      |     % --- 2. ПЕРЕИМЕНОВЫВАЕМ САМИ БЛОКИ (визуальные надписи UI0 -> UI1 и т.д.) ---
      |     % Ищем все элементы только внутри этой подсистемы
      |     internalBlocks = find_system(blockPath, 'SearchDepth', 1, 'LookUnderMasks', 'on');
      | 
      |     % Цикл начинаем с 2, так как 1-й элемент в списке - это сама папка подсистемы
      |     for i = 2:length(internalBlocks)
      |         oldName = get_param(internalBlocks{i}, 'Name');
      |         % Ищем цифру в конце имени и меняем на новую
      |         newName = regexprep(oldName, '\d+$', newNum);
      | 
      |         % Если имя изменилось, применяем его
      |         if ~strcmp(oldName, newName)
      |             try
      |                 set_param(internalBlocks{i}, 'Name', newName);
      |             catch
      |                 % Игнорируем ошибку, если вдруг такое имя уже случайно есть
      |             end
      |         end
      |     end
      | end
  M_IN_Город_5_4 : Subsystem
      settings: CopyFcn=|
      | % Получаем путь и имя нового (только что скопированного) блока
      | blockPath = gcb;
      | blockName = get_param(blockPath, 'Name');
      | 
      | % Ищем число в названии самой подсистемы (например, берем "2" из "Measure_2")
      | numStr = regexp(blockName, '\d+', 'match');
      | 
      | if ~isempty(numStr)
      |     newNum = numStr{end}; % Берем последнее найденное число
      | 
      |     % --- 1. Обновляем скрытые теги в Goto и From (радиочастоты) ---
      |     gotos = find_system(blockPath, 'LookUnderMasks', 'on', 'BlockType', 'Goto');
      |     froms = find_system(blockPath, 'LookUnderMasks', 'on', 'BlockType', 'From');
      | 
      |     for i = 1:length(gotos)
      |         oldTag = get_param(gotos{i}, 'GotoTag');
      |         set_param(gotos{i}, 'GotoTag', regexprep(oldTag, '\d+$', newNum));
      |     end
      |     for i = 1:length(froms)
      |         oldTag = get_param(froms{i}, 'GotoTag');
      |         set_param(froms{i}, 'GotoTag', regexprep(oldTag, '\d+$', newNum));
      |     end
      | 
      |     % --- 2. ПЕРЕИМЕНОВЫВАЕМ САМИ БЛОКИ (визуальные надписи UI0 -> UI1 и т.д.) ---
      |     % Ищем все элементы только внутри этой подсистемы
      |     internalBlocks = find_system(blockPath, 'SearchDepth', 1, 'LookUnderMasks', 'on');
      | 
      |     % Цикл начинаем с 2, так как 1-й элемент в списке - это сама папка подсистемы
      |     for i = 2:length(internalBlocks)
      |         oldName = get_param(internalBlocks{i}, 'Name');
      |         % Ищем цифру в конце имени и меняем на новую
      |         newName = regexprep(oldName, '\d+$', newNum);
      | 
      |         % Если имя изменилось, применяем его
      |         if ~strcmp(oldName, newName)
      |             try
      |                 set_param(internalBlocks{i}, 'Name', newName);
      |             catch
      |                 % Игнорируем ошибку, если вдруг такое имя уже случайно есть
      |             end
      |         end
      |     end
      | end
  M_IN_Город_6_1 : Subsystem
      settings: CopyFcn=|
      | % Получаем путь и имя нового (только что скопированного) блока
      | blockPath = gcb;
      | blockName = get_param(blockPath, 'Name');
      | 
      | % Ищем число в названии самой подсистемы (например, берем "2" из "Measure_2")
      | numStr = regexp(blockName, '\d+', 'match');
      | 
      | if ~isempty(numStr)
      |     newNum = numStr{end}; % Берем последнее найденное число
      | 
      |     % --- 1. Обновляем скрытые теги в Goto и From (радиочастоты) ---
      |     gotos = find_system(blockPath, 'LookUnderMasks', 'on', 'BlockType', 'Goto');
      |     froms = find_system(blockPath, 'LookUnderMasks', 'on', 'BlockType', 'From');
      | 
      |     for i = 1:length(gotos)
      |         oldTag = get_param(gotos{i}, 'GotoTag');
      |         set_param(gotos{i}, 'GotoTag', regexprep(oldTag, '\d+$', newNum));
      |     end
      |     for i = 1:length(froms)
      |         oldTag = get_param(froms{i}, 'GotoTag');
      |         set_param(froms{i}, 'GotoTag', regexprep(oldTag, '\d+$', newNum));
      |     end
      | 
      |     % --- 2. ПЕРЕИМЕНОВЫВАЕМ САМИ БЛОКИ (визуальные надписи UI0 -> UI1 и т.д.) ---
      |     % Ищем все элементы только внутри этой подсистемы
      |     internalBlocks = find_system(blockPath, 'SearchDepth', 1, 'LookUnderMasks', 'on');
      | 
      |     % Цикл начинаем с 2, так как 1-й элемент в списке - это сама папка подсистемы
      |     for i = 2:length(internalBlocks)
      |         oldName = get_param(internalBlocks{i}, 'Name');
      |         % Ищем цифру в конце имени и меняем на новую
      |         newName = regexprep(oldName, '\d+$', newNum);
      | 
      |         % Если имя изменилось, применяем его
      |         if ~strcmp(oldName, newName)
      |             try
      |                 set_param(internalBlocks{i}, 'Name', newName);
      |             catch
      |                 % Игнорируем ошибку, если вдруг такое имя уже случайно есть
      |             end
      |         end
      |     end
      | end
  M_IN_Город_6_2 : Subsystem
      settings: CopyFcn=|
      | % Получаем путь и имя нового (только что скопированного) блока
      | blockPath = gcb;
      | blockName = get_param(blockPath, 'Name');
      | 
      | % Ищем число в названии самой подсистемы (например, берем "2" из "Measure_2")
      | numStr = regexp(blockName, '\d+', 'match');
      | 
      | if ~isempty(numStr)
      |     newNum = numStr{end}; % Берем последнее найденное число
      | 
      |     % --- 1. Обновляем скрытые теги в Goto и From (радиочастоты) ---
      |     gotos = find_system(blockPath, 'LookUnderMasks', 'on', 'BlockType', 'Goto');
      |     froms = find_system(blockPath, 'LookUnderMasks', 'on', 'BlockType', 'From');
      | 
      |     for i = 1:length(gotos)
      |         oldTag = get_param(gotos{i}, 'GotoTag');
      |         set_param(gotos{i}, 'GotoTag', regexprep(oldTag, '\d+$', newNum));
      |     end
      |     for i = 1:length(froms)
      |         oldTag = get_param(froms{i}, 'GotoTag');
      |         set_param(froms{i}, 'GotoTag', regexprep(oldTag, '\d+$', newNum));
      |     end
      | 
      |     % --- 2. ПЕРЕИМЕНОВЫВАЕМ САМИ БЛОКИ (визуальные надписи UI0 -> UI1 и т.д.) ---
      |     % Ищем все элементы только внутри этой подсистемы
      |     internalBlocks = find_system(blockPath, 'SearchDepth', 1, 'LookUnderMasks', 'on');
      | 
      |     % Цикл начинаем с 2, так как 1-й элемент в списке - это сама папка подсистемы
      |     for i = 2:length(internalBlocks)
      |         oldName = get_param(internalBlocks{i}, 'Name');
      |         % Ищем цифру в конце имени и меняем на новую
      |         newName = regexprep(oldName, '\d+$', newNum);
      | 
      |         % Если имя изменилось, применяем его
      |         if ~strcmp(oldName, newName)
      |             try
      |                 set_param(internalBlocks{i}, 'Name', newName);
      |             catch
      |                 % Игнорируем ошибку, если вдруг такое имя уже случайно есть
      |             end
      |         end
      |     end
      | end
  M_IN_Город_6_3 : Subsystem
      settings: CopyFcn=|
      | % Получаем путь и имя нового (только что скопированного) блока
      | blockPath = gcb;
      | blockName = get_param(blockPath, 'Name');
      | 
      | % Ищем число в названии самой подсистемы (например, берем "2" из "Measure_2")
      | numStr = regexp(blockName, '\d+', 'match');
      | 
      | if ~isempty(numStr)
      |     newNum = numStr{end}; % Берем последнее найденное число
      | 
      |     % --- 1. Обновляем скрытые теги в Goto и From (радиочастоты) ---
      |     gotos = find_system(blockPath, 'LookUnderMasks', 'on', 'BlockType', 'Goto');
      |     froms = find_system(blockPath, 'LookUnderMasks', 'on', 'BlockType', 'From');
      | 
      |     for i = 1:length(gotos)
      |         oldTag = get_param(gotos{i}, 'GotoTag');
      |         set_param(gotos{i}, 'GotoTag', regexprep(oldTag, '\d+$', newNum));
      |     end
      |     for i = 1:length(froms)
      |         oldTag = get_param(froms{i}, 'GotoTag');
      |         set_param(froms{i}, 'GotoTag', regexprep(oldTag, '\d+$', newNum));
      |     end
      | 
      |     % --- 2. ПЕРЕИМЕНОВЫВАЕМ САМИ БЛОКИ (визуальные надписи UI0 -> UI1 и т.д.) ---
      |     % Ищем все элементы только внутри этой подсистемы
      |     internalBlocks = find_system(blockPath, 'SearchDepth', 1, 'LookUnderMasks', 'on');
      | 
      |     % Цикл начинаем с 2, так как 1-й элемент в списке - это сама папка подсистемы
      |     for i = 2:length(internalBlocks)
      |         oldName = get_param(internalBlocks{i}, 'Name');
      |         % Ищем цифру в конце имени и меняем на новую
      |         newName = regexprep(oldName, '\d+$', newNum);
      | 
      |         % Если имя изменилось, применяем его
      |         if ~strcmp(oldName, newName)
      |             try
      |                 set_param(internalBlocks{i}, 'Name', newName);
      |             catch
      |                 % Игнорируем ошибку, если вдруг такое имя уже случайно есть
      |             end
      |         end
      |     end
      | end
  M_IN_Город_6_4 : Subsystem
      settings: CopyFcn=|
      | % Получаем путь и имя нового (только что скопированного) блока
      | blockPath = gcb;
      | blockName = get_param(blockPath, 'Name');
      | 
      | % Ищем число в названии самой подсистемы (например, берем "2" из "Measure_2")
      | numStr = regexp(blockName, '\d+', 'match');
      | 
      | if ~isempty(numStr)
      |     newNum = numStr{end}; % Берем последнее найденное число
      | 
      |     % --- 1. Обновляем скрытые теги в Goto и From (радиочастоты) ---
      |     gotos = find_system(blockPath, 'LookUnderMasks', 'on', 'BlockType', 'Goto');
      |     froms = find_system(blockPath, 'LookUnderMasks', 'on', 'BlockType', 'From');
      | 
      |     for i = 1:length(gotos)
      |         oldTag = get_param(gotos{i}, 'GotoTag');
      |         set_param(gotos{i}, 'GotoTag', regexprep(oldTag, '\d+$', newNum));
      |     end
      |     for i = 1:length(froms)
      |         oldTag = get_param(froms{i}, 'GotoTag');
      |         set_param(froms{i}, 'GotoTag', regexprep(oldTag, '\d+$', newNum));
      |     end
      | 
      |     % --- 2. ПЕРЕИМЕНОВЫВАЕМ САМИ БЛОКИ (визуальные надписи UI0 -> UI1 и т.д.) ---
      |     % Ищем все элементы только внутри этой подсистемы
      |     internalBlocks = find_system(blockPath, 'SearchDepth', 1, 'LookUnderMasks', 'on');
      | 
      |     % Цикл начинаем с 2, так как 1-й элемент в списке - это сама папка подсистемы
      |     for i = 2:length(internalBlocks)
      |         oldName = get_param(internalBlocks{i}, 'Name');
      |         % Ищем цифру в конце имени и меняем на новую
      |         newName = regexprep(oldName, '\d+$', newNum);
      | 
      |         % Если имя изменилось, применяем его
      |         if ~strcmp(oldName, newName)
      |             try
      |                 set_param(internalBlocks{i}, 'Name', newName);
      |             catch
      |                 % Игнорируем ошибку, если вдруг такое имя уже случайно есть
      |             end
      |         end
      |     end
      | end
  M_IN_Завод_1_1 : Subsystem
      settings: CopyFcn=|
      | % Получаем путь и имя нового (только что скопированного) блока
      | blockPath = gcb;
      | blockName = get_param(blockPath, 'Name');
      | 
      | % Ищем число в названии самой подсистемы (например, берем "2" из "Measure_2")
      | numStr = regexp(blockName, '\d+', 'match');
      | 
      | if ~isempty(numStr)
      |     newNum = numStr{end}; % Берем последнее найденное число
      | 
      |     % --- 1. Обновляем скрытые теги в Goto и From (радиочастоты) ---
      |     gotos = find_system(blockPath, 'LookUnderMasks', 'on', 'BlockType', 'Goto');
      |     froms = find_system(blockPath, 'LookUnderMasks', 'on', 'BlockType', 'From');
      | 
      |     for i = 1:length(gotos)
      |         oldTag = get_param(gotos{i}, 'GotoTag');
      |         set_param(gotos{i}, 'GotoTag', regexprep(oldTag, '\d+$', newNum));
      |     end
      |     for i = 1:length(froms)
      |         oldTag = get_param(froms{i}, 'GotoTag');
      |         set_param(froms{i}, 'GotoTag', regexprep(oldTag, '\d+$', newNum));
      |     end
      | 
      |     % --- 2. ПЕРЕИМЕНОВЫВАЕМ САМИ БЛОКИ (визуальные надписи UI0 -> UI1 и т.д.) ---
      |     % Ищем все элементы только внутри этой подсистемы
      |     internalBlocks = find_system(blockPath, 'SearchDepth', 1, 'LookUnderMasks', 'on');
      | 
      |     % Цикл начинаем с 2, так как 1-й элемент в списке - это сама папка подсистемы
      |     for i = 2:length(internalBlocks)
      |         oldName = get_param(internalBlocks{i}, 'Name');
      |         % Ищем цифру в конце имени и меняем на новую
      |         newName = regexprep(oldName, '\d+$', newNum);
      | 
      |         % Если имя изменилось, применяем его
      |         if ~strcmp(oldName, newName)
      |             try
      |                 set_param(internalBlocks{i}, 'Name', newName);
      |             catch
      |                 % Игнорируем ошибку, если вдруг такое имя уже случайно есть
      |             end
      |         end
      |     end
      | end
  M_IN_Завод_1_2 : Subsystem
      settings: CopyFcn=|
      | % Получаем путь и имя нового (только что скопированного) блока
      | blockPath = gcb;
      | blockName = get_param(blockPath, 'Name');
      | 
      | % Ищем число в названии самой подсистемы (например, берем "2" из "Measure_2")
      | numStr = regexp(blockName, '\d+', 'match');
      | 
      | if ~isempty(numStr)
      |     newNum = numStr{end}; % Берем последнее найденное число
      | 
      |     % --- 1. Обновляем скрытые теги в Goto и From (радиочастоты) ---
      |     gotos = find_system(blockPath, 'LookUnderMasks', 'on', 'BlockType', 'Goto');
      |     froms = find_system(blockPath, 'LookUnderMasks', 'on', 'BlockType', 'From');
      | 
      |     for i = 1:length(gotos)
      |         oldTag = get_param(gotos{i}, 'GotoTag');
      |         set_param(gotos{i}, 'GotoTag', regexprep(oldTag, '\d+$', newNum));
      |     end
      |     for i = 1:length(froms)
      |         oldTag = get_param(froms{i}, 'GotoTag');
      |         set_param(froms{i}, 'GotoTag', regexprep(oldTag, '\d+$', newNum));
      |     end
      | 
      |     % --- 2. ПЕРЕИМЕНОВЫВАЕМ САМИ БЛОКИ (визуальные надписи UI0 -> UI1 и т.д.) ---
      |     % Ищем все элементы только внутри этой подсистемы
      |     internalBlocks = find_system(blockPath, 'SearchDepth', 1, 'LookUnderMasks', 'on');
      | 
      |     % Цикл начинаем с 2, так как 1-й элемент в списке - это сама папка подсистемы
      |     for i = 2:length(internalBlocks)
      |         oldName = get_param(internalBlocks{i}, 'Name');
      |         % Ищем цифру в конце имени и меняем на новую
      |         newName = regexprep(oldName, '\d+$', newNum);
      | 
      |         % Если имя изменилось, применяем его
      |         if ~strcmp(oldName, newName)
      |             try
      |                 set_param(internalBlocks{i}, 'Name', newName);
      |             catch
      |                 % Игнорируем ошибку, если вдруг такое имя уже случайно есть
      |             end
      |         end
      |     end
      | end
  M_IN_Завод_2_1 : Subsystem
      settings: CopyFcn=|
      | % Получаем путь и имя нового (только что скопированного) блока
      | blockPath = gcb;
      | blockName = get_param(blockPath, 'Name');
      | 
      | % Ищем число в названии самой подсистемы (например, берем "2" из "Measure_2")
      | numStr = regexp(blockName, '\d+', 'match');
      | 
      | if ~isempty(numStr)
      |     newNum = numStr{end}; % Берем последнее найденное число
      | 
      |     % --- 1. Обновляем скрытые теги в Goto и From (радиочастоты) ---
      |     gotos = find_system(blockPath, 'LookUnderMasks', 'on', 'BlockType', 'Goto');
      |     froms = find_system(blockPath, 'LookUnderMasks', 'on', 'BlockType', 'From');
      | 
      |     for i = 1:length(gotos)
      |         oldTag = get_param(gotos{i}, 'GotoTag');
      |         set_param(gotos{i}, 'GotoTag', regexprep(oldTag, '\d+$', newNum));
      |     end
      |     for i = 1:length(froms)
      |         oldTag = get_param(froms{i}, 'GotoTag');
      |         set_param(froms{i}, 'GotoTag', regexprep(oldTag, '\d+$', newNum));
      |     end
      | 
      |     % --- 2. ПЕРЕИМЕНОВЫВАЕМ САМИ БЛОКИ (визуальные надписи UI0 -> UI1 и т.д.) ---
      |     % Ищем все элементы только внутри этой подсистемы
      |     internalBlocks = find_system(blockPath, 'SearchDepth', 1, 'LookUnderMasks', 'on');
      | 
      |     % Цикл начинаем с 2, так как 1-й элемент в списке - это сама папка подсистемы
      |     for i = 2:length(internalBlocks)
      |         oldName = get_param(internalBlocks{i}, 'Name');
      |         % Ищем цифру в конце имени и меняем на новую
      |         newName = regexprep(oldName, '\d+$', newNum);
      | 
      |         % Если имя изменилось, применяем его
      |         if ~strcmp(oldName, newName)
      |             try
      |                 set_param(internalBlocks{i}, 'Name', newName);
      |             catch
      |                 % Игнорируем ошибку, если вдруг такое имя уже случайно есть
      |             end
      |         end
      |     end
      | end
  M_IN_Завод_2_2 : Subsystem
      settings: CopyFcn=|
      | % Получаем путь и имя нового (только что скопированного) блока
      | blockPath = gcb;
      | blockName = get_param(blockPath, 'Name');
      | 
      | % Ищем число в названии самой подсистемы (например, берем "2" из "Measure_2")
      | numStr = regexp(blockName, '\d+', 'match');
      | 
      | if ~isempty(numStr)
      |     newNum = numStr{end}; % Берем последнее найденное число
      | 
      |     % --- 1. Обновляем скрытые теги в Goto и From (радиочастоты) ---
      |     gotos = find_system(blockPath, 'LookUnderMasks', 'on', 'BlockType', 'Goto');
      |     froms = find_system(blockPath, 'LookUnderMasks', 'on', 'BlockType', 'From');
      | 
      |     for i = 1:length(gotos)
      |         oldTag = get_param(gotos{i}, 'GotoTag');
      |         set_param(gotos{i}, 'GotoTag', regexprep(oldTag, '\d+$', newNum));
      |     end
      |     for i = 1:length(froms)
      |         oldTag = get_param(froms{i}, 'GotoTag');
      |         set_param(froms{i}, 'GotoTag', regexprep(oldTag, '\d+$', newNum));
      |     end
      | 
      |     % --- 2. ПЕРЕИМЕНОВЫВАЕМ САМИ БЛОКИ (визуальные надписи UI0 -> UI1 и т.д.) ---
      |     % Ищем все элементы только внутри этой подсистемы
      |     internalBlocks = find_system(blockPath, 'SearchDepth', 1, 'LookUnderMasks', 'on');
      | 
      |     % Цикл начинаем с 2, так как 1-й элемент в списке - это сама папка подсистемы
      |     for i = 2:length(internalBlocks)
      |         oldName = get_param(internalBlocks{i}, 'Name');
      |         % Ищем цифру в конце имени и меняем на новую
      |         newName = regexprep(oldName, '\d+$', newNum);
      | 
      |         % Если имя изменилось, применяем его
      |         if ~strcmp(oldName, newName)
      |             try
      |                 set_param(internalBlocks{i}, 'Name', newName);
      |             catch
      |                 % Игнорируем ошибку, если вдруг такое имя уже случайно есть
      |             end
      |         end
      |     end
      | end
  M_IN_Завод_3_1 : Subsystem
      settings: CopyFcn=|
      | % Получаем путь и имя нового (только что скопированного) блока
      | blockPath = gcb;
      | blockName = get_param(blockPath, 'Name');
      | 
      | % Ищем число в названии самой подсистемы (например, берем "2" из "Measure_2")
      | numStr = regexp(blockName, '\d+', 'match');
      | 
      | if ~isempty(numStr)
      |     newNum = numStr{end}; % Берем последнее найденное число
      | 
      |     % --- 1. Обновляем скрытые теги в Goto и From (радиочастоты) ---
      |     gotos = find_system(blockPath, 'LookUnderMasks', 'on', 'BlockType', 'Goto');
      |     froms = find_system(blockPath, 'LookUnderMasks', 'on', 'BlockType', 'From');
      | 
      |     for i = 1:length(gotos)
      |         oldTag = get_param(gotos{i}, 'GotoTag');
      |         set_param(gotos{i}, 'GotoTag', regexprep(oldTag, '\d+$', newNum));
      |     end
      |     for i = 1:length(froms)
      |         oldTag = get_param(froms{i}, 'GotoTag');
      |         set_param(froms{i}, 'GotoTag', regexprep(oldTag, '\d+$', newNum));
      |     end
      | 
      |     % --- 2. ПЕРЕИМЕНОВЫВАЕМ САМИ БЛОКИ (визуальные надписи UI0 -> UI1 и т.д.) ---
      |     % Ищем все элементы только внутри этой подсистемы
      |     internalBlocks = find_system(blockPath, 'SearchDepth', 1, 'LookUnderMasks', 'on');
      | 
      |     % Цикл начинаем с 2, так как 1-й элемент в списке - это сама папка подсистемы
      |     for i = 2:length(internalBlocks)
      |         oldName = get_param(internalBlocks{i}, 'Name');
      |         % Ищем цифру в конце имени и меняем на новую
      |         newName = regexprep(oldName, '\d+$', newNum);
      | 
      |         % Если имя изменилось, применяем его
      |         if ~strcmp(oldName, newName)
      |             try
      |                 set_param(internalBlocks{i}, 'Name', newName);
      |             catch
      |                 % Игнорируем ошибку, если вдруг такое имя уже случайно есть
      |             end
      |         end
      |     end
      | end
  M_IN_Завод_3_2 : Subsystem
      settings: CopyFcn=|
      | % Получаем путь и имя нового (только что скопированного) блока
      | blockPath = gcb;
      | blockName = get_param(blockPath, 'Name');
      | 
      | % Ищем число в названии самой подсистемы (например, берем "2" из "Measure_2")
      | numStr = regexp(blockName, '\d+', 'match');
      | 
      | if ~isempty(numStr)
      |     newNum = numStr{end}; % Берем последнее найденное число
      | 
      |     % --- 1. Обновляем скрытые теги в Goto и From (радиочастоты) ---
      |     gotos = find_system(blockPath, 'LookUnderMasks', 'on', 'BlockType', 'Goto');
      |     froms = find_system(blockPath, 'LookUnderMasks', 'on', 'BlockType', 'From');
      | 
      |     for i = 1:length(gotos)
      |         oldTag = get_param(gotos{i}, 'GotoTag');
      |         set_param(gotos{i}, 'GotoTag', regexprep(oldTag, '\d+$', newNum));
      |     end
      |     for i = 1:length(froms)
      |         oldTag = get_param(froms{i}, 'GotoTag');
      |         set_param(froms{i}, 'GotoTag', regexprep(oldTag, '\d+$', newNum));
      |     end
      | 
      |     % --- 2. ПЕРЕИМЕНОВЫВАЕМ САМИ БЛОКИ (визуальные надписи UI0 -> UI1 и т.д.) ---
      |     % Ищем все элементы только внутри этой подсистемы
      |     internalBlocks = find_system(blockPath, 'SearchDepth', 1, 'LookUnderMasks', 'on');
      | 
      |     % Цикл начинаем с 2, так как 1-й элемент в списке - это сама папка подсистемы
      |     for i = 2:length(internalBlocks)
      |         oldName = get_param(internalBlocks{i}, 'Name');
      |         % Ищем цифру в конце имени и меняем на новую
      |         newName = regexprep(oldName, '\d+$', newNum);
      | 
      |         % Если имя изменилось, применяем его
      |         if ~strcmp(oldName, newName)
      |             try
      |                 set_param(internalBlocks{i}, 'Name', newName);
      |             catch
      |                 % Игнорируем ошибку, если вдруг такое имя уже случайно есть
      |             end
      |         end
      |     end
      | end
  M_IN_Завод_4_1 : Subsystem
      settings: CopyFcn=|
      | % Получаем путь и имя нового (только что скопированного) блока
      | blockPath = gcb;
      | blockName = get_param(blockPath, 'Name');
      | 
      | % Ищем число в названии самой подсистемы (например, берем "2" из "Measure_2")
      | numStr = regexp(blockName, '\d+', 'match');
      | 
      | if ~isempty(numStr)
      |     newNum = numStr{end}; % Берем последнее найденное число
      | 
      |     % --- 1. Обновляем скрытые теги в Goto и From (радиочастоты) ---
      |     gotos = find_system(blockPath, 'LookUnderMasks', 'on', 'BlockType', 'Goto');
      |     froms = find_system(blockPath, 'LookUnderMasks', 'on', 'BlockType', 'From');
      | 
      |     for i = 1:length(gotos)
      |         oldTag = get_param(gotos{i}, 'GotoTag');
      |         set_param(gotos{i}, 'GotoTag', regexprep(oldTag, '\d+$', newNum));
      |     end
      |     for i = 1:length(froms)
      |         oldTag = get_param(froms{i}, 'GotoTag');
      |         set_param(froms{i}, 'GotoTag', regexprep(oldTag, '\d+$', newNum));
      |     end
      | 
      |     % --- 2. ПЕРЕИМЕНОВЫВАЕМ САМИ БЛОКИ (визуальные надписи UI0 -> UI1 и т.д.) ---
      |     % Ищем все элементы только внутри этой подсистемы
      |     internalBlocks = find_system(blockPath, 'SearchDepth', 1, 'LookUnderMasks', 'on');
      | 
      |     % Цикл начинаем с 2, так как 1-й элемент в списке - это сама папка подсистемы
      |     for i = 2:length(internalBlocks)
      |         oldName = get_param(internalBlocks{i}, 'Name');
      |         % Ищем цифру в конце имени и меняем на новую
      |         newName = regexprep(oldName, '\d+$', newNum);
      | 
      |         % Если имя изменилось, применяем его
      |         if ~strcmp(oldName, newName)
      |             try
      |                 set_param(internalBlocks{i}, 'Name', newName);
      |             catch
      |                 % Игнорируем ошибку, если вдруг такое имя уже случайно есть
      |             end
      |         end
      |     end
      | end
  M_IN_Завод_4_2 : Subsystem
      settings: CopyFcn=|
      | % Получаем путь и имя нового (только что скопированного) блока
      | blockPath = gcb;
      | blockName = get_param(blockPath, 'Name');
      | 
      | % Ищем число в названии самой подсистемы (например, берем "2" из "Measure_2")
      | numStr = regexp(blockName, '\d+', 'match');
      | 
      | if ~isempty(numStr)
      |     newNum = numStr{end}; % Берем последнее найденное число
      | 
      |     % --- 1. Обновляем скрытые теги в Goto и From (радиочастоты) ---
      |     gotos = find_system(blockPath, 'LookUnderMasks', 'on', 'BlockType', 'Goto');
      |     froms = find_system(blockPath, 'LookUnderMasks', 'on', 'BlockType', 'From');
      | 
      |     for i = 1:length(gotos)
      |         oldTag = get_param(gotos{i}, 'GotoTag');
      |         set_param(gotos{i}, 'GotoTag', regexprep(oldTag, '\d+$', newNum));
      |     end
      |     for i = 1:length(froms)
      |         oldTag = get_param(froms{i}, 'GotoTag');
      |         set_param(froms{i}, 'GotoTag', regexprep(oldTag, '\d+$', newNum));
      |     end
      | 
      |     % --- 2. ПЕРЕИМЕНОВЫВАЕМ САМИ БЛОКИ (визуальные надписи UI0 -> UI1 и т.д.) ---
      |     % Ищем все элементы только внутри этой подсистемы
      |     internalBlocks = find_system(blockPath, 'SearchDepth', 1, 'LookUnderMasks', 'on');
      | 
      |     % Цикл начинаем с 2, так как 1-й элемент в списке - это сама папка подсистемы
      |     for i = 2:length(internalBlocks)
      |         oldName = get_param(internalBlocks{i}, 'Name');
      |         % Ищем цифру в конце имени и меняем на новую
      |         newName = regexprep(oldName, '\d+$', newNum);
      | 
      |         % Если имя изменилось, применяем его
      |         if ~strcmp(oldName, newName)
      |             try
      |                 set_param(internalBlocks{i}, 'Name', newName);
      |             catch
      |                 % Игнорируем ошибку, если вдруг такое имя уже случайно есть
      |             end
      |         end
      |     end
      | end
  M_IN_Завод_5_1 : Subsystem
      settings: CopyFcn=|
      | % Получаем путь и имя нового (только что скопированного) блока
      | blockPath = gcb;
      | blockName = get_param(blockPath, 'Name');
      | 
      | % Ищем число в названии самой подсистемы (например, берем "2" из "Measure_2")
      | numStr = regexp(blockName, '\d+', 'match');
      | 
      | if ~isempty(numStr)
      |     newNum = numStr{end}; % Берем последнее найденное число
      | 
      |     % --- 1. Обновляем скрытые теги в Goto и From (радиочастоты) ---
      |     gotos = find_system(blockPath, 'LookUnderMasks', 'on', 'BlockType', 'Goto');
      |     froms = find_system(blockPath, 'LookUnderMasks', 'on', 'BlockType', 'From');
      | 
      |     for i = 1:length(gotos)
      |         oldTag = get_param(gotos{i}, 'GotoTag');
      |         set_param(gotos{i}, 'GotoTag', regexprep(oldTag, '\d+$', newNum));
      |     end
      |     for i = 1:length(froms)
      |         oldTag = get_param(froms{i}, 'GotoTag');
      |         set_param(froms{i}, 'GotoTag', regexprep(oldTag, '\d+$', newNum));
      |     end
      | 
      |     % --- 2. ПЕРЕИМЕНОВЫВАЕМ САМИ БЛОКИ (визуальные надписи UI0 -> UI1 и т.д.) ---
      |     % Ищем все элементы только внутри этой подсистемы
      |     internalBlocks = find_system(blockPath, 'SearchDepth', 1, 'LookUnderMasks', 'on');
      | 
      |     % Цикл начинаем с 2, так как 1-й элемент в списке - это сама папка подсистемы
      |     for i = 2:length(internalBlocks)
      |         oldName = get_param(internalBlocks{i}, 'Name');
      |         % Ищем цифру в конце имени и меняем на новую
      |         newName = regexprep(oldName, '\d+$', newNum);
      | 
      |         % Если имя изменилось, применяем его
      |         if ~strcmp(oldName, newName)
      |             try
      |                 set_param(internalBlocks{i}, 'Name', newName);
      |             catch
      |                 % Игнорируем ошибку, если вдруг такое имя уже случайно есть
      |             end
      |         end
      |     end
      | end
  M_IN_Завод_5_2 : Subsystem
      settings: CopyFcn=|
      | % Получаем путь и имя нового (только что скопированного) блока
      | blockPath = gcb;
      | blockName = get_param(blockPath, 'Name');
      | 
      | % Ищем число в названии самой подсистемы (например, берем "2" из "Measure_2")
      | numStr = regexp(blockName, '\d+', 'match');
      | 
      | if ~isempty(numStr)
      |     newNum = numStr{end}; % Берем последнее найденное число
      | 
      |     % --- 1. Обновляем скрытые теги в Goto и From (радиочастоты) ---
      |     gotos = find_system(blockPath, 'LookUnderMasks', 'on', 'BlockType', 'Goto');
      |     froms = find_system(blockPath, 'LookUnderMasks', 'on', 'BlockType', 'From');
      | 
      |     for i = 1:length(gotos)
      |         oldTag = get_param(gotos{i}, 'GotoTag');
      |         set_param(gotos{i}, 'GotoTag', regexprep(oldTag, '\d+$', newNum));
      |     end
      |     for i = 1:length(froms)
      |         oldTag = get_param(froms{i}, 'GotoTag');
      |         set_param(froms{i}, 'GotoTag', regexprep(oldTag, '\d+$', newNum));
      |     end
      | 
      |     % --- 2. ПЕРЕИМЕНОВЫВАЕМ САМИ БЛОКИ (визуальные надписи UI0 -> UI1 и т.д.) ---
      |     % Ищем все элементы только внутри этой подсистемы
      |     internalBlocks = find_system(blockPath, 'SearchDepth', 1, 'LookUnderMasks', 'on');
      | 
      |     % Цикл начинаем с 2, так как 1-й элемент в списке - это сама папка подсистемы
      |     for i = 2:length(internalBlocks)
      |         oldName = get_param(internalBlocks{i}, 'Name');
      |         % Ищем цифру в конце имени и меняем на новую
      |         newName = regexprep(oldName, '\d+$', newNum);
      | 
      |         % Если имя изменилось, применяем его
      |         if ~strcmp(oldName, newName)
      |             try
      |                 set_param(internalBlocks{i}, 'Name', newName);
      |             catch
      |                 % Игнорируем ошибку, если вдруг такое имя уже случайно есть
      |             end
      |         end
      |     end
      | end
  M_IN_Завод_6_1 : Subsystem
      settings: CopyFcn=|
      | % Получаем путь и имя нового (только что скопированного) блока
      | blockPath = gcb;
      | blockName = get_param(blockPath, 'Name');
      | 
      | % Ищем число в названии самой подсистемы (например, берем "2" из "Measure_2")
      | numStr = regexp(blockName, '\d+', 'match');
      | 
      | if ~isempty(numStr)
      |     newNum = numStr{end}; % Берем последнее найденное число
      | 
      |     % --- 1. Обновляем скрытые теги в Goto и From (радиочастоты) ---
      |     gotos = find_system(blockPath, 'LookUnderMasks', 'on', 'BlockType', 'Goto');
      |     froms = find_system(blockPath, 'LookUnderMasks', 'on', 'BlockType', 'From');
      | 
      |     for i = 1:length(gotos)
      |         oldTag = get_param(gotos{i}, 'GotoTag');
      |         set_param(gotos{i}, 'GotoTag', regexprep(oldTag, '\d+$', newNum));
      |     end
      |     for i = 1:length(froms)
      |         oldTag = get_param(froms{i}, 'GotoTag');
      |         set_param(froms{i}, 'GotoTag', regexprep(oldTag, '\d+$', newNum));
      |     end
      | 
      |     % --- 2. ПЕРЕИМЕНОВЫВАЕМ САМИ БЛОКИ (визуальные надписи UI0 -> UI1 и т.д.) ---
      |     % Ищем все элементы только внутри этой подсистемы
      |     internalBlocks = find_system(blockPath, 'SearchDepth', 1, 'LookUnderMasks', 'on');
      | 
      |     % Цикл начинаем с 2, так как 1-й элемент в списке - это сама папка подсистемы
      |     for i = 2:length(internalBlocks)
      |         oldName = get_param(internalBlocks{i}, 'Name');
      |         % Ищем цифру в конце имени и меняем на новую
      |         newName = regexprep(oldName, '\d+$', newNum);
      | 
      |         % Если имя изменилось, применяем его
      |         if ~strcmp(oldName, newName)
      |             try
      |                 set_param(internalBlocks{i}, 'Name', newName);
      |             catch
      |                 % Игнорируем ошибку, если вдруг такое имя уже случайно есть
      |             end
      |         end
      |     end
      | end
  M_IN_Завод_6_2 : Subsystem
      settings: CopyFcn=|
      | % Получаем путь и имя нового (только что скопированного) блока
      | blockPath = gcb;
      | blockName = get_param(blockPath, 'Name');
      | 
      | % Ищем число в названии самой подсистемы (например, берем "2" из "Measure_2")
      | numStr = regexp(blockName, '\d+', 'match');
      | 
      | if ~isempty(numStr)
      |     newNum = numStr{end}; % Берем последнее найденное число
      | 
      |     % --- 1. Обновляем скрытые теги в Goto и From (радиочастоты) ---
      |     gotos = find_system(blockPath, 'LookUnderMasks', 'on', 'BlockType', 'Goto');
      |     froms = find_system(blockPath, 'LookUnderMasks', 'on', 'BlockType', 'From');
      | 
      |     for i = 1:length(gotos)
      |         oldTag = get_param(gotos{i}, 'GotoTag');
      |         set_param(gotos{i}, 'GotoTag', regexprep(oldTag, '\d+$', newNum));
      |     end
      |     for i = 1:length(froms)
      |         oldTag = get_param(froms{i}, 'GotoTag');
      |         set_param(froms{i}, 'GotoTag', regexprep(oldTag, '\d+$', newNum));
      |     end
      | 
      |     % --- 2. ПЕРЕИМЕНОВЫВАЕМ САМИ БЛОКИ (визуальные надписи UI0 -> UI1 и т.д.) ---
      |     % Ищем все элементы только внутри этой подсистемы
      |     internalBlocks = find_system(blockPath, 'SearchDepth', 1, 'LookUnderMasks', 'on');
      | 
      |     % Цикл начинаем с 2, так как 1-й элемент в списке - это сама папка подсистемы
      |     for i = 2:length(internalBlocks)
      |         oldName = get_param(internalBlocks{i}, 'Name');
      |         % Ищем цифру в конце имени и меняем на новую
      |         newName = regexprep(oldName, '\d+$', newNum);
      | 
      |         % Если имя изменилось, применяем его
      |         if ~strcmp(oldName, newName)
      |             try
      |                 set_param(internalBlocks{i}, 'Name', newName);
      |             catch
      |                 % Игнорируем ошибку, если вдруг такое имя уже случайно есть
      |             end
      |         end
      |     end
      | end
  M_OUT_Город_1_1 : Subsystem
      settings: CopyFcn=|
      | % Получаем путь и имя нового (только что скопированного) блока
      | blockPath = gcb;
      | blockName = get_param(blockPath, 'Name');
      | 
      | % Ищем число в названии самой подсистемы (например, берем "2" из "Measure_2")
      | numStr = regexp(blockName, '\d+', 'match');
      | 
      | if ~isempty(numStr)
      |     newNum = numStr{end}; % Берем последнее найденное число
      | 
      |     % --- 1. Обновляем скрытые теги в Goto и From (радиочастоты) ---
      |     gotos = find_system(blockPath, 'LookUnderMasks', 'on', 'BlockType', 'Goto');
      |     froms = find_system(blockPath, 'LookUnderMasks', 'on', 'BlockType', 'From');
      | 
      |     for i = 1:length(gotos)
      |         oldTag = get_param(gotos{i}, 'GotoTag');
      |         set_param(gotos{i}, 'GotoTag', regexprep(oldTag, '\d+$', newNum));
      |     end
      |     for i = 1:length(froms)
      |         oldTag = get_param(froms{i}, 'GotoTag');
      |         set_param(froms{i}, 'GotoTag', regexprep(oldTag, '\d+$', newNum));
      |     end
      | 
      |     % --- 2. ПЕРЕИМЕНОВЫВАЕМ САМИ БЛОКИ (визуальные надписи UI0 -> UI1 и т.д.) ---
      |     % Ищем все элементы только внутри этой подсистемы
      |     internalBlocks = find_system(blockPath, 'SearchDepth', 1, 'LookUnderMasks', 'on');
      | 
      |     % Цикл начинаем с 2, так как 1-й элемент в списке - это сама папка подсистемы
      |     for i = 2:length(internalBlocks)
      |         oldName = get_param(internalBlocks{i}, 'Name');
      |         % Ищем цифру в конце имени и меняем на новую
      |         newName = regexprep(oldName, '\d+$', newNum);
      | 
      |         % Если имя изменилось, применяем его
      |         if ~strcmp(oldName, newName)
      |             try
      |                 set_param(internalBlocks{i}, 'Name', newName);
      |             catch
      |                 % Игнорируем ошибку, если вдруг такое имя уже случайно есть
      |             end
      |         end
      |     end
      | end
  M_OUT_Город_1_2 : Subsystem
      settings: CopyFcn=|
      | % Получаем путь и имя нового (только что скопированного) блока
      | blockPath = gcb;
      | blockName = get_param(blockPath, 'Name');
      | 
      | % Ищем число в названии самой подсистемы (например, берем "2" из "Measure_2")
      | numStr = regexp(blockName, '\d+', 'match');
      | 
      | if ~isempty(numStr)
      |     newNum = numStr{end}; % Берем последнее найденное число
      | 
      |     % --- 1. Обновляем скрытые теги в Goto и From (радиочастоты) ---
      |     gotos = find_system(blockPath, 'LookUnderMasks', 'on', 'BlockType', 'Goto');
      |     froms = find_system(blockPath, 'LookUnderMasks', 'on', 'BlockType', 'From');
      | 
      |     for i = 1:length(gotos)
      |         oldTag = get_param(gotos{i}, 'GotoTag');
      |         set_param(gotos{i}, 'GotoTag', regexprep(oldTag, '\d+$', newNum));
      |     end
      |     for i = 1:length(froms)
      |         oldTag = get_param(froms{i}, 'GotoTag');
      |         set_param(froms{i}, 'GotoTag', regexprep(oldTag, '\d+$', newNum));
      |     end
      | 
      |     % --- 2. ПЕРЕИМЕНОВЫВАЕМ САМИ БЛОКИ (визуальные надписи UI0 -> UI1 и т.д.) ---
      |     % Ищем все элементы только внутри этой подсистемы
      |     internalBlocks = find_system(blockPath, 'SearchDepth', 1, 'LookUnderMasks', 'on');
      | 
      |     % Цикл начинаем с 2, так как 1-й элемент в списке - это сама папка подсистемы
      |     for i = 2:length(internalBlocks)
      |         oldName = get_param(internalBlocks{i}, 'Name');
      |         % Ищем цифру в конце имени и меняем на новую
      |         newName = regexprep(oldName, '\d+$', newNum);
      | 
      |         % Если имя изменилось, применяем его
      |         if ~strcmp(oldName, newName)
      |             try
      |                 set_param(internalBlocks{i}, 'Name', newName);
      |             catch
      |                 % Игнорируем ошибку, если вдруг такое имя уже случайно есть
      |             end
      |         end
      |     end
      | end
  M_OUT_Город_1_3 : Subsystem
      settings: CopyFcn=|
      | % Получаем путь и имя нового (только что скопированного) блока
      | blockPath = gcb;
      | blockName = get_param(blockPath, 'Name');
      | 
      | % Ищем число в названии самой подсистемы (например, берем "2" из "Measure_2")
      | numStr = regexp(blockName, '\d+', 'match');
      | 
      | if ~isempty(numStr)
      |     newNum = numStr{end}; % Берем последнее найденное число
      | 
      |     % --- 1. Обновляем скрытые теги в Goto и From (радиочастоты) ---
      |     gotos = find_system(blockPath, 'LookUnderMasks', 'on', 'BlockType', 'Goto');
      |     froms = find_system(blockPath, 'LookUnderMasks', 'on', 'BlockType', 'From');
      | 
      |     for i = 1:length(gotos)
      |         oldTag = get_param(gotos{i}, 'GotoTag');
      |         set_param(gotos{i}, 'GotoTag', regexprep(oldTag, '\d+$', newNum));
      |     end
      |     for i = 1:length(froms)
      |         oldTag = get_param(froms{i}, 'GotoTag');
      |         set_param(froms{i}, 'GotoTag', regexprep(oldTag, '\d+$', newNum));
      |     end
      | 
      |     % --- 2. ПЕРЕИМЕНОВЫВАЕМ САМИ БЛОКИ (визуальные надписи UI0 -> UI1 и т.д.) ---
      |     % Ищем все элементы только внутри этой подсистемы
      |     internalBlocks = find_system(blockPath, 'SearchDepth', 1, 'LookUnderMasks', 'on');
      | 
      |     % Цикл начинаем с 2, так как 1-й элемент в списке - это сама папка подсистемы
      |     for i = 2:length(internalBlocks)
      |         oldName = get_param(internalBlocks{i}, 'Name');
      |         % Ищем цифру в конце имени и меняем на новую
      |         newName = regexprep(oldName, '\d+$', newNum);
      | 
      |         % Если имя изменилось, применяем его
      |         if ~strcmp(oldName, newName)
      |             try
      |                 set_param(internalBlocks{i}, 'Name', newName);
      |             catch
      |                 % Игнорируем ошибку, если вдруг такое имя уже случайно есть
      |             end
      |         end
      |     end
      | end
  M_OUT_Город_1_4 : Subsystem
      settings: CopyFcn=|
      | % Получаем путь и имя нового (только что скопированного) блока
      | blockPath = gcb;
      | blockName = get_param(blockPath, 'Name');
      | 
      | % Ищем число в названии самой подсистемы (например, берем "2" из "Measure_2")
      | numStr = regexp(blockName, '\d+', 'match');
      | 
      | if ~isempty(numStr)
      |     newNum = numStr{end}; % Берем последнее найденное число
      | 
      |     % --- 1. Обновляем скрытые теги в Goto и From (радиочастоты) ---
      |     gotos = find_system(blockPath, 'LookUnderMasks', 'on', 'BlockType', 'Goto');
      |     froms = find_system(blockPath, 'LookUnderMasks', 'on', 'BlockType', 'From');
      | 
      |     for i = 1:length(gotos)
      |         oldTag = get_param(gotos{i}, 'GotoTag');
      |         set_param(gotos{i}, 'GotoTag', regexprep(oldTag, '\d+$', newNum));
      |     end
      |     for i = 1:length(froms)
      |         oldTag = get_param(froms{i}, 'GotoTag');
      |         set_param(froms{i}, 'GotoTag', regexprep(oldTag, '\d+$', newNum));
      |     end
      | 
      |     % --- 2. ПЕРЕИМЕНОВЫВАЕМ САМИ БЛОКИ (визуальные надписи UI0 -> UI1 и т.д.) ---
      |     % Ищем все элементы только внутри этой подсистемы
      |     internalBlocks = find_system(blockPath, 'SearchDepth', 1, 'LookUnderMasks', 'on');
      | 
      |     % Цикл начинаем с 2, так как 1-й элемент в списке - это сама папка подсистемы
      |     for i = 2:length(internalBlocks)
      |         oldName = get_param(internalBlocks{i}, 'Name');
      |         % Ищем цифру в конце имени и меняем на новую
      |         newName = regexprep(oldName, '\d+$', newNum);
      | 
      |         % Если имя изменилось, применяем его
      |         if ~strcmp(oldName, newName)
      |             try
      |                 set_param(internalBlocks{i}, 'Name', newName);
      |             catch
      |                 % Игнорируем ошибку, если вдруг такое имя уже случайно есть
      |             end
      |         end
      |     end
      | end
  M_OUT_Город_2_1 : Subsystem
      settings: CopyFcn=|
      | % Получаем путь и имя нового (только что скопированного) блока
      | blockPath = gcb;
      | blockName = get_param(blockPath, 'Name');
      | 
      | % Ищем число в названии самой подсистемы (например, берем "2" из "Measure_2")
      | numStr = regexp(blockName, '\d+', 'match');
      | 
      | if ~isempty(numStr)
      |     newNum = numStr{end}; % Берем последнее найденное число
      | 
      |     % --- 1. Обновляем скрытые теги в Goto и From (радиочастоты) ---
      |     gotos = find_system(blockPath, 'LookUnderMasks', 'on', 'BlockType', 'Goto');
      |     froms = find_system(blockPath, 'LookUnderMasks', 'on', 'BlockType', 'From');
      | 
      |     for i = 1:length(gotos)
      |         oldTag = get_param(gotos{i}, 'GotoTag');
      |         set_param(gotos{i}, 'GotoTag', regexprep(oldTag, '\d+$', newNum));
      |     end
      |     for i = 1:length(froms)
      |         oldTag = get_param(froms{i}, 'GotoTag');
      |         set_param(froms{i}, 'GotoTag', regexprep(oldTag, '\d+$', newNum));
      |     end
      | 
      |     % --- 2. ПЕРЕИМЕНОВЫВАЕМ САМИ БЛОКИ (визуальные надписи UI0 -> UI1 и т.д.) ---
      |     % Ищем все элементы только внутри этой подсистемы
      |     internalBlocks = find_system(blockPath, 'SearchDepth', 1, 'LookUnderMasks', 'on');
      | 
      |     % Цикл начинаем с 2, так как 1-й элемент в списке - это сама папка подсистемы
      |     for i = 2:length(internalBlocks)
      |         oldName = get_param(internalBlocks{i}, 'Name');
      |         % Ищем цифру в конце имени и меняем на новую
      |         newName = regexprep(oldName, '\d+$', newNum);
      | 
      |         % Если имя изменилось, применяем его
      |         if ~strcmp(oldName, newName)
      |             try
      |                 set_param(internalBlocks{i}, 'Name', newName);
      |             catch
      |                 % Игнорируем ошибку, если вдруг такое имя уже случайно есть
      |             end
      |         end
      |     end
      | end
  M_OUT_Город_2_2 : Subsystem
      settings: CopyFcn=|
      | % Получаем путь и имя нового (только что скопированного) блока
      | blockPath = gcb;
      | blockName = get_param(blockPath, 'Name');
      | 
      | % Ищем число в названии самой подсистемы (например, берем "2" из "Measure_2")
      | numStr = regexp(blockName, '\d+', 'match');
      | 
      | if ~isempty(numStr)
      |     newNum = numStr{end}; % Берем последнее найденное число
      | 
      |     % --- 1. Обновляем скрытые теги в Goto и From (радиочастоты) ---
      |     gotos = find_system(blockPath, 'LookUnderMasks', 'on', 'BlockType', 'Goto');
      |     froms = find_system(blockPath, 'LookUnderMasks', 'on', 'BlockType', 'From');
      | 
      |     for i = 1:length(gotos)
      |         oldTag = get_param(gotos{i}, 'GotoTag');
      |         set_param(gotos{i}, 'GotoTag', regexprep(oldTag, '\d+$', newNum));
      |     end
      |     for i = 1:length(froms)
      |         oldTag = get_param(froms{i}, 'GotoTag');
      |         set_param(froms{i}, 'GotoTag', regexprep(oldTag, '\d+$', newNum));
      |     end
      | 
      |     % --- 2. ПЕРЕИМЕНОВЫВАЕМ САМИ БЛОКИ (визуальные надписи UI0 -> UI1 и т.д.) ---
      |     % Ищем все элементы только внутри этой подсистемы
      |     internalBlocks = find_system(blockPath, 'SearchDepth', 1, 'LookUnderMasks', 'on');
      | 
      |     % Цикл начинаем с 2, так как 1-й элемент в списке - это сама папка подсистемы
      |     for i = 2:length(internalBlocks)
      |         oldName = get_param(internalBlocks{i}, 'Name');
      |         % Ищем цифру в конце имени и меняем на новую
      |         newName = regexprep(oldName, '\d+$', newNum);
      | 
      |         % Если имя изменилось, применяем его
      |         if ~strcmp(oldName, newName)
      |             try
      |                 set_param(internalBlocks{i}, 'Name', newName);
      |             catch
      |                 % Игнорируем ошибку, если вдруг такое имя уже случайно есть
      |             end
      |         end
      |     end
      | end
  M_OUT_Город_2_3 : Subsystem
      settings: CopyFcn=|
      | % Получаем путь и имя нового (только что скопированного) блока
      | blockPath = gcb;
      | blockName = get_param(blockPath, 'Name');
      | 
      | % Ищем число в названии самой подсистемы (например, берем "2" из "Measure_2")
      | numStr = regexp(blockName, '\d+', 'match');
      | 
      | if ~isempty(numStr)
      |     newNum = numStr{end}; % Берем последнее найденное число
      | 
      |     % --- 1. Обновляем скрытые теги в Goto и From (радиочастоты) ---
      |     gotos = find_system(blockPath, 'LookUnderMasks', 'on', 'BlockType', 'Goto');
      |     froms = find_system(blockPath, 'LookUnderMasks', 'on', 'BlockType', 'From');
      | 
      |     for i = 1:length(gotos)
      |         oldTag = get_param(gotos{i}, 'GotoTag');
      |         set_param(gotos{i}, 'GotoTag', regexprep(oldTag, '\d+$', newNum));
      |     end
      |     for i = 1:length(froms)
      |         oldTag = get_param(froms{i}, 'GotoTag');
      |         set_param(froms{i}, 'GotoTag', regexprep(oldTag, '\d+$', newNum));
      |     end
      | 
      |     % --- 2. ПЕРЕИМЕНОВЫВАЕМ САМИ БЛОКИ (визуальные надписи UI0 -> UI1 и т.д.) ---
      |     % Ищем все элементы только внутри этой подсистемы
      |     internalBlocks = find_system(blockPath, 'SearchDepth', 1, 'LookUnderMasks', 'on');
      | 
      |     % Цикл начинаем с 2, так как 1-й элемент в списке - это сама папка подсистемы
      |     for i = 2:length(internalBlocks)
      |         oldName = get_param(internalBlocks{i}, 'Name');
      |         % Ищем цифру в конце имени и меняем на новую
      |         newName = regexprep(oldName, '\d+$', newNum);
      | 
      |         % Если имя изменилось, применяем его
      |         if ~strcmp(oldName, newName)
      |             try
      |                 set_param(internalBlocks{i}, 'Name', newName);
      |             catch
      |                 % Игнорируем ошибку, если вдруг такое имя уже случайно есть
      |             end
      |         end
      |     end
      | end
  M_OUT_Город_2_4 : Subsystem
      settings: CopyFcn=|
      | % Получаем путь и имя нового (только что скопированного) блока
      | blockPath = gcb;
      | blockName = get_param(blockPath, 'Name');
      | 
      | % Ищем число в названии самой подсистемы (например, берем "2" из "Measure_2")
      | numStr = regexp(blockName, '\d+', 'match');
      | 
      | if ~isempty(numStr)
      |     newNum = numStr{end}; % Берем последнее найденное число
      | 
      |     % --- 1. Обновляем скрытые теги в Goto и From (радиочастоты) ---
      |     gotos = find_system(blockPath, 'LookUnderMasks', 'on', 'BlockType', 'Goto');
      |     froms = find_system(blockPath, 'LookUnderMasks', 'on', 'BlockType', 'From');
      | 
      |     for i = 1:length(gotos)
      |         oldTag = get_param(gotos{i}, 'GotoTag');
      |         set_param(gotos{i}, 'GotoTag', regexprep(oldTag, '\d+$', newNum));
      |     end
      |     for i = 1:length(froms)
      |         oldTag = get_param(froms{i}, 'GotoTag');
      |         set_param(froms{i}, 'GotoTag', regexprep(oldTag, '\d+$', newNum));
      |     end
      | 
      |     % --- 2. ПЕРЕИМЕНОВЫВАЕМ САМИ БЛОКИ (визуальные надписи UI0 -> UI1 и т.д.) ---
      |     % Ищем все элементы только внутри этой подсистемы
      |     internalBlocks = find_system(blockPath, 'SearchDepth', 1, 'LookUnderMasks', 'on');
      | 
      |     % Цикл начинаем с 2, так как 1-й элемент в списке - это сама папка подсистемы
      |     for i = 2:length(internalBlocks)
      |         oldName = get_param(internalBlocks{i}, 'Name');
      |         % Ищем цифру в конце имени и меняем на новую
      |         newName = regexprep(oldName, '\d+$', newNum);
      | 
      |         % Если имя изменилось, применяем его
      |         if ~strcmp(oldName, newName)
      |             try
      |                 set_param(internalBlocks{i}, 'Name', newName);
      |             catch
      |                 % Игнорируем ошибку, если вдруг такое имя уже случайно есть
      |             end
      |         end
      |     end
      | end
  M_OUT_Город_3_1 : Subsystem
      settings: CopyFcn=|
      | % Получаем путь и имя нового (только что скопированного) блока
      | blockPath = gcb;
      | blockName = get_param(blockPath, 'Name');
      | 
      | % Ищем число в названии самой подсистемы (например, берем "2" из "Measure_2")
      | numStr = regexp(blockName, '\d+', 'match');
      | 
      | if ~isempty(numStr)
      |     newNum = numStr{end}; % Берем последнее найденное число
      | 
      |     % --- 1. Обновляем скрытые теги в Goto и From (радиочастоты) ---
      |     gotos = find_system(blockPath, 'LookUnderMasks', 'on', 'BlockType', 'Goto');
      |     froms = find_system(blockPath, 'LookUnderMasks', 'on', 'BlockType', 'From');
      | 
      |     for i = 1:length(gotos)
      |         oldTag = get_param(gotos{i}, 'GotoTag');
      |         set_param(gotos{i}, 'GotoTag', regexprep(oldTag, '\d+$', newNum));
      |     end
      |     for i = 1:length(froms)
      |         oldTag = get_param(froms{i}, 'GotoTag');
      |         set_param(froms{i}, 'GotoTag', regexprep(oldTag, '\d+$', newNum));
      |     end
      | 
      |     % --- 2. ПЕРЕИМЕНОВЫВАЕМ САМИ БЛОКИ (визуальные надписи UI0 -> UI1 и т.д.) ---
      |     % Ищем все элементы только внутри этой подсистемы
      |     internalBlocks = find_system(blockPath, 'SearchDepth', 1, 'LookUnderMasks', 'on');
      | 
      |     % Цикл начинаем с 2, так как 1-й элемент в списке - это сама папка подсистемы
      |     for i = 2:length(internalBlocks)
      |         oldName = get_param(internalBlocks{i}, 'Name');
      |         % Ищем цифру в конце имени и меняем на новую
      |         newName = regexprep(oldName, '\d+$', newNum);
      | 
      |         % Если имя изменилось, применяем его
      |         if ~strcmp(oldName, newName)
      |             try
      |                 set_param(internalBlocks{i}, 'Name', newName);
      |             catch
      |                 % Игнорируем ошибку, если вдруг такое имя уже случайно есть
      |             end
      |         end
      |     end
      | end
  M_OUT_Город_3_2 : Subsystem
      settings: CopyFcn=|
      | % Получаем путь и имя нового (только что скопированного) блока
      | blockPath = gcb;
      | blockName = get_param(blockPath, 'Name');
      | 
      | % Ищем число в названии самой подсистемы (например, берем "2" из "Measure_2")
      | numStr = regexp(blockName, '\d+', 'match');
      | 
      | if ~isempty(numStr)
      |     newNum = numStr{end}; % Берем последнее найденное число
      | 
      |     % --- 1. Обновляем скрытые теги в Goto и From (радиочастоты) ---
      |     gotos = find_system(blockPath, 'LookUnderMasks', 'on', 'BlockType', 'Goto');
      |     froms = find_system(blockPath, 'LookUnderMasks', 'on', 'BlockType', 'From');
      | 
      |     for i = 1:length(gotos)
      |         oldTag = get_param(gotos{i}, 'GotoTag');
      |         set_param(gotos{i}, 'GotoTag', regexprep(oldTag, '\d+$', newNum));
      |     end
      |     for i = 1:length(froms)
      |         oldTag = get_param(froms{i}, 'GotoTag');
      |         set_param(froms{i}, 'GotoTag', regexprep(oldTag, '\d+$', newNum));
      |     end
      | 
      |     % --- 2. ПЕРЕИМЕНОВЫВАЕМ САМИ БЛОКИ (визуальные надписи UI0 -> UI1 и т.д.) ---
      |     % Ищем все элементы только внутри этой подсистемы
      |     internalBlocks = find_system(blockPath, 'SearchDepth', 1, 'LookUnderMasks', 'on');
      | 
      |     % Цикл начинаем с 2, так как 1-й элемент в списке - это сама папка подсистемы
      |     for i = 2:length(internalBlocks)
      |         oldName = get_param(internalBlocks{i}, 'Name');
      |         % Ищем цифру в конце имени и меняем на новую
      |         newName = regexprep(oldName, '\d+$', newNum);
      | 
      |         % Если имя изменилось, применяем его
      |         if ~strcmp(oldName, newName)
      |             try
      |                 set_param(internalBlocks{i}, 'Name', newName);
      |             catch
      |                 % Игнорируем ошибку, если вдруг такое имя уже случайно есть
      |             end
      |         end
      |     end
      | end
  M_OUT_Город_3_3 : Subsystem
      settings: CopyFcn=|
      | % Получаем путь и имя нового (только что скопированного) блока
      | blockPath = gcb;
      | blockName = get_param(blockPath, 'Name');
      | 
      | % Ищем число в названии самой подсистемы (например, берем "2" из "Measure_2")
      | numStr = regexp(blockName, '\d+', 'match');
      | 
      | if ~isempty(numStr)
      |     newNum = numStr{end}; % Берем последнее найденное число
      | 
      |     % --- 1. Обновляем скрытые теги в Goto и From (радиочастоты) ---
      |     gotos = find_system(blockPath, 'LookUnderMasks', 'on', 'BlockType', 'Goto');
      |     froms = find_system(blockPath, 'LookUnderMasks', 'on', 'BlockType', 'From');
      | 
      |     for i = 1:length(gotos)
      |         oldTag = get_param(gotos{i}, 'GotoTag');
      |         set_param(gotos{i}, 'GotoTag', regexprep(oldTag, '\d+$', newNum));
      |     end
      |     for i = 1:length(froms)
      |         oldTag = get_param(froms{i}, 'GotoTag');
      |         set_param(froms{i}, 'GotoTag', regexprep(oldTag, '\d+$', newNum));
      |     end
      | 
      |     % --- 2. ПЕРЕИМЕНОВЫВАЕМ САМИ БЛОКИ (визуальные надписи UI0 -> UI1 и т.д.) ---
      |     % Ищем все элементы только внутри этой подсистемы
      |     internalBlocks = find_system(blockPath, 'SearchDepth', 1, 'LookUnderMasks', 'on');
      | 
      |     % Цикл начинаем с 2, так как 1-й элемент в списке - это сама папка подсистемы
      |     for i = 2:length(internalBlocks)
      |         oldName = get_param(internalBlocks{i}, 'Name');
      |         % Ищем цифру в конце имени и меняем на новую
      |         newName = regexprep(oldName, '\d+$', newNum);
      | 
      |         % Если имя изменилось, применяем его
      |         if ~strcmp(oldName, newName)
      |             try
      |                 set_param(internalBlocks{i}, 'Name', newName);
      |             catch
      |                 % Игнорируем ошибку, если вдруг такое имя уже случайно есть
      |             end
      |         end
      |     end
      | end
  M_OUT_Город_3_4 : Subsystem
      settings: CopyFcn=|
      | % Получаем путь и имя нового (только что скопированного) блока
      | blockPath = gcb;
      | blockName = get_param(blockPath, 'Name');
      | 
      | % Ищем число в названии самой подсистемы (например, берем "2" из "Measure_2")
      | numStr = regexp(blockName, '\d+', 'match');
      | 
      | if ~isempty(numStr)
      |     newNum = numStr{end}; % Берем последнее найденное число
      | 
      |     % --- 1. Обновляем скрытые теги в Goto и From (радиочастоты) ---
      |     gotos = find_system(blockPath, 'LookUnderMasks', 'on', 'BlockType', 'Goto');
      |     froms = find_system(blockPath, 'LookUnderMasks', 'on', 'BlockType', 'From');
      | 
      |     for i = 1:length(gotos)
      |         oldTag = get_param(gotos{i}, 'GotoTag');
      |         set_param(gotos{i}, 'GotoTag', regexprep(oldTag, '\d+$', newNum));
      |     end
      |     for i = 1:length(froms)
      |         oldTag = get_param(froms{i}, 'GotoTag');
      |         set_param(froms{i}, 'GotoTag', regexprep(oldTag, '\d+$', newNum));
      |     end
      | 
      |     % --- 2. ПЕРЕИМЕНОВЫВАЕМ САМИ БЛОКИ (визуальные надписи UI0 -> UI1 и т.д.) ---
      |     % Ищем все элементы только внутри этой подсистемы
      |     internalBlocks = find_system(blockPath, 'SearchDepth', 1, 'LookUnderMasks', 'on');
      | 
      |     % Цикл начинаем с 2, так как 1-й элемент в списке - это сама папка подсистемы
      |     for i = 2:length(internalBlocks)
      |         oldName = get_param(internalBlocks{i}, 'Name');
      |         % Ищем цифру в конце имени и меняем на новую
      |         newName = regexprep(oldName, '\d+$', newNum);
      | 
      |         % Если имя изменилось, применяем его
      |         if ~strcmp(oldName, newName)
      |             try
      |                 set_param(internalBlocks{i}, 'Name', newName);
      |             catch
      |                 % Игнорируем ошибку, если вдруг такое имя уже случайно есть
      |             end
      |         end
      |     end
      | end
  M_OUT_Город_4_1 : Subsystem
      settings: CopyFcn=|
      | % Получаем путь и имя нового (только что скопированного) блока
      | blockPath = gcb;
      | blockName = get_param(blockPath, 'Name');
      | 
      | % Ищем число в названии самой подсистемы (например, берем "2" из "Measure_2")
      | numStr = regexp(blockName, '\d+', 'match');
      | 
      | if ~isempty(numStr)
      |     newNum = numStr{end}; % Берем последнее найденное число
      | 
      |     % --- 1. Обновляем скрытые теги в Goto и From (радиочастоты) ---
      |     gotos = find_system(blockPath, 'LookUnderMasks', 'on', 'BlockType', 'Goto');
      |     froms = find_system(blockPath, 'LookUnderMasks', 'on', 'BlockType', 'From');
      | 
      |     for i = 1:length(gotos)
      |         oldTag = get_param(gotos{i}, 'GotoTag');
      |         set_param(gotos{i}, 'GotoTag', regexprep(oldTag, '\d+$', newNum));
      |     end
      |     for i = 1:length(froms)
      |         oldTag = get_param(froms{i}, 'GotoTag');
      |         set_param(froms{i}, 'GotoTag', regexprep(oldTag, '\d+$', newNum));
      |     end
      | 
      |     % --- 2. ПЕРЕИМЕНОВЫВАЕМ САМИ БЛОКИ (визуальные надписи UI0 -> UI1 и т.д.) ---
      |     % Ищем все элементы только внутри этой подсистемы
      |     internalBlocks = find_system(blockPath, 'SearchDepth', 1, 'LookUnderMasks', 'on');
      | 
      |     % Цикл начинаем с 2, так как 1-й элемент в списке - это сама папка подсистемы
      |     for i = 2:length(internalBlocks)
      |         oldName = get_param(internalBlocks{i}, 'Name');
      |         % Ищем цифру в конце имени и меняем на новую
      |         newName = regexprep(oldName, '\d+$', newNum);
      | 
      |         % Если имя изменилось, применяем его
      |         if ~strcmp(oldName, newName)
      |             try
      |                 set_param(internalBlocks{i}, 'Name', newName);
      |             catch
      |                 % Игнорируем ошибку, если вдруг такое имя уже случайно есть
      |             end
      |         end
      |     end
      | end
  M_OUT_Город_4_2 : Subsystem
      settings: CopyFcn=|
      | % Получаем путь и имя нового (только что скопированного) блока
      | blockPath = gcb;
      | blockName = get_param(blockPath, 'Name');
      | 
      | % Ищем число в названии самой подсистемы (например, берем "2" из "Measure_2")
      | numStr = regexp(blockName, '\d+', 'match');
      | 
      | if ~isempty(numStr)
      |     newNum = numStr{end}; % Берем последнее найденное число
      | 
      |     % --- 1. Обновляем скрытые теги в Goto и From (радиочастоты) ---
      |     gotos = find_system(blockPath, 'LookUnderMasks', 'on', 'BlockType', 'Goto');
      |     froms = find_system(blockPath, 'LookUnderMasks', 'on', 'BlockType', 'From');
      | 
      |     for i = 1:length(gotos)
      |         oldTag = get_param(gotos{i}, 'GotoTag');
      |         set_param(gotos{i}, 'GotoTag', regexprep(oldTag, '\d+$', newNum));
      |     end
      |     for i = 1:length(froms)
      |         oldTag = get_param(froms{i}, 'GotoTag');
      |         set_param(froms{i}, 'GotoTag', regexprep(oldTag, '\d+$', newNum));
      |     end
      | 
      |     % --- 2. ПЕРЕИМЕНОВЫВАЕМ САМИ БЛОКИ (визуальные надписи UI0 -> UI1 и т.д.) ---
      |     % Ищем все элементы только внутри этой подсистемы
      |     internalBlocks = find_system(blockPath, 'SearchDepth', 1, 'LookUnderMasks', 'on');
      | 
      |     % Цикл начинаем с 2, так как 1-й элемент в списке - это сама папка подсистемы
      |     for i = 2:length(internalBlocks)
      |         oldName = get_param(internalBlocks{i}, 'Name');
      |         % Ищем цифру в конце имени и меняем на новую
      |         newName = regexprep(oldName, '\d+$', newNum);
      | 
      |         % Если имя изменилось, применяем его
      |         if ~strcmp(oldName, newName)
      |             try
      |                 set_param(internalBlocks{i}, 'Name', newName);
      |             catch
      |                 % Игнорируем ошибку, если вдруг такое имя уже случайно есть
      |             end
      |         end
      |     end
      | end
  M_OUT_Город_4_3 : Subsystem
      settings: CopyFcn=|
      | % Получаем путь и имя нового (только что скопированного) блока
      | blockPath = gcb;
      | blockName = get_param(blockPath, 'Name');
      | 
      | % Ищем число в названии самой подсистемы (например, берем "2" из "Measure_2")
      | numStr = regexp(blockName, '\d+', 'match');
      | 
      | if ~isempty(numStr)
      |     newNum = numStr{end}; % Берем последнее найденное число
      | 
      |     % --- 1. Обновляем скрытые теги в Goto и From (радиочастоты) ---
      |     gotos = find_system(blockPath, 'LookUnderMasks', 'on', 'BlockType', 'Goto');
      |     froms = find_system(blockPath, 'LookUnderMasks', 'on', 'BlockType', 'From');
      | 
      |     for i = 1:length(gotos)
      |         oldTag = get_param(gotos{i}, 'GotoTag');
      |         set_param(gotos{i}, 'GotoTag', regexprep(oldTag, '\d+$', newNum));
      |     end
      |     for i = 1:length(froms)
      |         oldTag = get_param(froms{i}, 'GotoTag');
      |         set_param(froms{i}, 'GotoTag', regexprep(oldTag, '\d+$', newNum));
      |     end
      | 
      |     % --- 2. ПЕРЕИМЕНОВЫВАЕМ САМИ БЛОКИ (визуальные надписи UI0 -> UI1 и т.д.) ---
      |     % Ищем все элементы только внутри этой подсистемы
      |     internalBlocks = find_system(blockPath, 'SearchDepth', 1, 'LookUnderMasks', 'on');
      | 
      |     % Цикл начинаем с 2, так как 1-й элемент в списке - это сама папка подсистемы
      |     for i = 2:length(internalBlocks)
      |         oldName = get_param(internalBlocks{i}, 'Name');
      |         % Ищем цифру в конце имени и меняем на новую
      |         newName = regexprep(oldName, '\d+$', newNum);
      | 
      |         % Если имя изменилось, применяем его
      |         if ~strcmp(oldName, newName)
      |             try
      |                 set_param(internalBlocks{i}, 'Name', newName);
      |             catch
      |                 % Игнорируем ошибку, если вдруг такое имя уже случайно есть
      |             end
      |         end
      |     end
      | end
  M_OUT_Город_4_4 : Subsystem
      settings: CopyFcn=|
      | % Получаем путь и имя нового (только что скопированного) блока
      | blockPath = gcb;
      | blockName = get_param(blockPath, 'Name');
      | 
      | % Ищем число в названии самой подсистемы (например, берем "2" из "Measure_2")
      | numStr = regexp(blockName, '\d+', 'match');
      | 
      | if ~isempty(numStr)
      |     newNum = numStr{end}; % Берем последнее найденное число
      | 
      |     % --- 1. Обновляем скрытые теги в Goto и From (радиочастоты) ---
      |     gotos = find_system(blockPath, 'LookUnderMasks', 'on', 'BlockType', 'Goto');
      |     froms = find_system(blockPath, 'LookUnderMasks', 'on', 'BlockType', 'From');
      | 
      |     for i = 1:length(gotos)
      |         oldTag = get_param(gotos{i}, 'GotoTag');
      |         set_param(gotos{i}, 'GotoTag', regexprep(oldTag, '\d+$', newNum));
      |     end
      |     for i = 1:length(froms)
      |         oldTag = get_param(froms{i}, 'GotoTag');
      |         set_param(froms{i}, 'GotoTag', regexprep(oldTag, '\d+$', newNum));
      |     end
      | 
      |     % --- 2. ПЕРЕИМЕНОВЫВАЕМ САМИ БЛОКИ (визуальные надписи UI0 -> UI1 и т.д.) ---
      |     % Ищем все элементы только внутри этой подсистемы
      |     internalBlocks = find_system(blockPath, 'SearchDepth', 1, 'LookUnderMasks', 'on');
      | 
      |     % Цикл начинаем с 2, так как 1-й элемент в списке - это сама папка подсистемы
      |     for i = 2:length(internalBlocks)
      |         oldName = get_param(internalBlocks{i}, 'Name');
      |         % Ищем цифру в конце имени и меняем на новую
      |         newName = regexprep(oldName, '\d+$', newNum);
      | 
      |         % Если имя изменилось, применяем его
      |         if ~strcmp(oldName, newName)
      |             try
      |                 set_param(internalBlocks{i}, 'Name', newName);
      |             catch
      |                 % Игнорируем ошибку, если вдруг такое имя уже случайно есть
      |             end
      |         end
      |     end
      | end
  M_OUT_Город_5_1 : Subsystem
      settings: CopyFcn=|
      | % Получаем путь и имя нового (только что скопированного) блока
      | blockPath = gcb;
      | blockName = get_param(blockPath, 'Name');
      | 
      | % Ищем число в названии самой подсистемы (например, берем "2" из "Measure_2")
      | numStr = regexp(blockName, '\d+', 'match');
      | 
      | if ~isempty(numStr)
      |     newNum = numStr{end}; % Берем последнее найденное число
      | 
      |     % --- 1. Обновляем скрытые теги в Goto и From (радиочастоты) ---
      |     gotos = find_system(blockPath, 'LookUnderMasks', 'on', 'BlockType', 'Goto');
      |     froms = find_system(blockPath, 'LookUnderMasks', 'on', 'BlockType', 'From');
      | 
      |     for i = 1:length(gotos)
      |         oldTag = get_param(gotos{i}, 'GotoTag');
      |         set_param(gotos{i}, 'GotoTag', regexprep(oldTag, '\d+$', newNum));
      |     end
      |     for i = 1:length(froms)
      |         oldTag = get_param(froms{i}, 'GotoTag');
      |         set_param(froms{i}, 'GotoTag', regexprep(oldTag, '\d+$', newNum));
      |     end
      | 
      |     % --- 2. ПЕРЕИМЕНОВЫВАЕМ САМИ БЛОКИ (визуальные надписи UI0 -> UI1 и т.д.) ---
      |     % Ищем все элементы только внутри этой подсистемы
      |     internalBlocks = find_system(blockPath, 'SearchDepth', 1, 'LookUnderMasks', 'on');
      | 
      |     % Цикл начинаем с 2, так как 1-й элемент в списке - это сама папка подсистемы
      |     for i = 2:length(internalBlocks)
      |         oldName = get_param(internalBlocks{i}, 'Name');
      |         % Ищем цифру в конце имени и меняем на новую
      |         newName = regexprep(oldName, '\d+$', newNum);
      | 
      |         % Если имя изменилось, применяем его
      |         if ~strcmp(oldName, newName)
      |             try
      |                 set_param(internalBlocks{i}, 'Name', newName);
      |             catch
      |                 % Игнорируем ошибку, если вдруг такое имя уже случайно есть
      |             end
      |         end
      |     end
      | end
  M_OUT_Город_5_2 : Subsystem
      settings: CopyFcn=|
      | % Получаем путь и имя нового (только что скопированного) блока
      | blockPath = gcb;
      | blockName = get_param(blockPath, 'Name');
      | 
      | % Ищем число в названии самой подсистемы (например, берем "2" из "Measure_2")
      | numStr = regexp(blockName, '\d+', 'match');
      | 
      | if ~isempty(numStr)
      |     newNum = numStr{end}; % Берем последнее найденное число
      | 
      |     % --- 1. Обновляем скрытые теги в Goto и From (радиочастоты) ---
      |     gotos = find_system(blockPath, 'LookUnderMasks', 'on', 'BlockType', 'Goto');
      |     froms = find_system(blockPath, 'LookUnderMasks', 'on', 'BlockType', 'From');
      | 
      |     for i = 1:length(gotos)
      |         oldTag = get_param(gotos{i}, 'GotoTag');
      |         set_param(gotos{i}, 'GotoTag', regexprep(oldTag, '\d+$', newNum));
      |     end
      |     for i = 1:length(froms)
      |         oldTag = get_param(froms{i}, 'GotoTag');
      |         set_param(froms{i}, 'GotoTag', regexprep(oldTag, '\d+$', newNum));
      |     end
      | 
      |     % --- 2. ПЕРЕИМЕНОВЫВАЕМ САМИ БЛОКИ (визуальные надписи UI0 -> UI1 и т.д.) ---
      |     % Ищем все элементы только внутри этой подсистемы
      |     internalBlocks = find_system(blockPath, 'SearchDepth', 1, 'LookUnderMasks', 'on');
      | 
      |     % Цикл начинаем с 2, так как 1-й элемент в списке - это сама папка подсистемы
      |     for i = 2:length(internalBlocks)
      |         oldName = get_param(internalBlocks{i}, 'Name');
      |         % Ищем цифру в конце имени и меняем на новую
      |         newName = regexprep(oldName, '\d+$', newNum);
      | 
      |         % Если имя изменилось, применяем его
      |         if ~strcmp(oldName, newName)
      |             try
      |                 set_param(internalBlocks{i}, 'Name', newName);
      |             catch
      |                 % Игнорируем ошибку, если вдруг такое имя уже случайно есть
      |             end
      |         end
      |     end
      | end
  M_OUT_Город_5_3 : Subsystem
      settings: CopyFcn=|
      | % Получаем путь и имя нового (только что скопированного) блока
      | blockPath = gcb;
      | blockName = get_param(blockPath, 'Name');
      | 
      | % Ищем число в названии самой подсистемы (например, берем "2" из "Measure_2")
      | numStr = regexp(blockName, '\d+', 'match');
      | 
      | if ~isempty(numStr)
      |     newNum = numStr{end}; % Берем последнее найденное число
      | 
      |     % --- 1. Обновляем скрытые теги в Goto и From (радиочастоты) ---
      |     gotos = find_system(blockPath, 'LookUnderMasks', 'on', 'BlockType', 'Goto');
      |     froms = find_system(blockPath, 'LookUnderMasks', 'on', 'BlockType', 'From');
      | 
      |     for i = 1:length(gotos)
      |         oldTag = get_param(gotos{i}, 'GotoTag');
      |         set_param(gotos{i}, 'GotoTag', regexprep(oldTag, '\d+$', newNum));
      |     end
      |     for i = 1:length(froms)
      |         oldTag = get_param(froms{i}, 'GotoTag');
      |         set_param(froms{i}, 'GotoTag', regexprep(oldTag, '\d+$', newNum));
      |     end
      | 
      |     % --- 2. ПЕРЕИМЕНОВЫВАЕМ САМИ БЛОКИ (визуальные надписи UI0 -> UI1 и т.д.) ---
      |     % Ищем все элементы только внутри этой подсистемы
      |     internalBlocks = find_system(blockPath, 'SearchDepth', 1, 'LookUnderMasks', 'on');
      | 
      |     % Цикл начинаем с 2, так как 1-й элемент в списке - это сама папка подсистемы
      |     for i = 2:length(internalBlocks)
      |         oldName = get_param(internalBlocks{i}, 'Name');
      |         % Ищем цифру в конце имени и меняем на новую
      |         newName = regexprep(oldName, '\d+$', newNum);
      | 
      |         % Если имя изменилось, применяем его
      |         if ~strcmp(oldName, newName)
      |             try
      |                 set_param(internalBlocks{i}, 'Name', newName);
      |             catch
      |                 % Игнорируем ошибку, если вдруг такое имя уже случайно есть
      |             end
      |         end
      |     end
      | end
  M_OUT_Город_5_4 : Subsystem
      settings: CopyFcn=|
      | % Получаем путь и имя нового (только что скопированного) блока
      | blockPath = gcb;
      | blockName = get_param(blockPath, 'Name');
      | 
      | % Ищем число в названии самой подсистемы (например, берем "2" из "Measure_2")
      | numStr = regexp(blockName, '\d+', 'match');
      | 
      | if ~isempty(numStr)
      |     newNum = numStr{end}; % Берем последнее найденное число
      | 
      |     % --- 1. Обновляем скрытые теги в Goto и From (радиочастоты) ---
      |     gotos = find_system(blockPath, 'LookUnderMasks', 'on', 'BlockType', 'Goto');
      |     froms = find_system(blockPath, 'LookUnderMasks', 'on', 'BlockType', 'From');
      | 
      |     for i = 1:length(gotos)
      |         oldTag = get_param(gotos{i}, 'GotoTag');
      |         set_param(gotos{i}, 'GotoTag', regexprep(oldTag, '\d+$', newNum));
      |     end
      |     for i = 1:length(froms)
      |         oldTag = get_param(froms{i}, 'GotoTag');
      |         set_param(froms{i}, 'GotoTag', regexprep(oldTag, '\d+$', newNum));
      |     end
      | 
      |     % --- 2. ПЕРЕИМЕНОВЫВАЕМ САМИ БЛОКИ (визуальные надписи UI0 -> UI1 и т.д.) ---
      |     % Ищем все элементы только внутри этой подсистемы
      |     internalBlocks = find_system(blockPath, 'SearchDepth', 1, 'LookUnderMasks', 'on');
      | 
      |     % Цикл начинаем с 2, так как 1-й элемент в списке - это сама папка подсистемы
      |     for i = 2:length(internalBlocks)
      |         oldName = get_param(internalBlocks{i}, 'Name');
      |         % Ищем цифру в конце имени и меняем на новую
      |         newName = regexprep(oldName, '\d+$', newNum);
      | 
      |         % Если имя изменилось, применяем его
      |         if ~strcmp(oldName, newName)
      |             try
      |                 set_param(internalBlocks{i}, 'Name', newName);
      |             catch
      |                 % Игнорируем ошибку, если вдруг такое имя уже случайно есть
      |             end
      |         end
      |     end
      | end
  M_OUT_Город_6_1 : Subsystem
      settings: CopyFcn=|
      | % Получаем путь и имя нового (только что скопированного) блока
      | blockPath = gcb;
      | blockName = get_param(blockPath, 'Name');
      | 
      | % Ищем число в названии самой подсистемы (например, берем "2" из "Measure_2")
      | numStr = regexp(blockName, '\d+', 'match');
      | 
      | if ~isempty(numStr)
      |     newNum = numStr{end}; % Берем последнее найденное число
      | 
      |     % --- 1. Обновляем скрытые теги в Goto и From (радиочастоты) ---
      |     gotos = find_system(blockPath, 'LookUnderMasks', 'on', 'BlockType', 'Goto');
      |     froms = find_system(blockPath, 'LookUnderMasks', 'on', 'BlockType', 'From');
      | 
      |     for i = 1:length(gotos)
      |         oldTag = get_param(gotos{i}, 'GotoTag');
      |         set_param(gotos{i}, 'GotoTag', regexprep(oldTag, '\d+$', newNum));
      |     end
      |     for i = 1:length(froms)
      |         oldTag = get_param(froms{i}, 'GotoTag');
      |         set_param(froms{i}, 'GotoTag', regexprep(oldTag, '\d+$', newNum));
      |     end
      | 
      |     % --- 2. ПЕРЕИМЕНОВЫВАЕМ САМИ БЛОКИ (визуальные надписи UI0 -> UI1 и т.д.) ---
      |     % Ищем все элементы только внутри этой подсистемы
      |     internalBlocks = find_system(blockPath, 'SearchDepth', 1, 'LookUnderMasks', 'on');
      | 
      |     % Цикл начинаем с 2, так как 1-й элемент в списке - это сама папка подсистемы
      |     for i = 2:length(internalBlocks)
      |         oldName = get_param(internalBlocks{i}, 'Name');
      |         % Ищем цифру в конце имени и меняем на новую
      |         newName = regexprep(oldName, '\d+$', newNum);
      | 
      |         % Если имя изменилось, применяем его
      |         if ~strcmp(oldName, newName)
      |             try
      |                 set_param(internalBlocks{i}, 'Name', newName);
      |             catch
      |                 % Игнорируем ошибку, если вдруг такое имя уже случайно есть
      |             end
      |         end
      |     end
      | end
  M_OUT_Город_6_2 : Subsystem
      settings: CopyFcn=|
      | % Получаем путь и имя нового (только что скопированного) блока
      | blockPath = gcb;
      | blockName = get_param(blockPath, 'Name');
      | 
      | % Ищем число в названии самой подсистемы (например, берем "2" из "Measure_2")
      | numStr = regexp(blockName, '\d+', 'match');
      | 
      | if ~isempty(numStr)
      |     newNum = numStr{end}; % Берем последнее найденное число
      | 
      |     % --- 1. Обновляем скрытые теги в Goto и From (радиочастоты) ---
      |     gotos = find_system(blockPath, 'LookUnderMasks', 'on', 'BlockType', 'Goto');
      |     froms = find_system(blockPath, 'LookUnderMasks', 'on', 'BlockType', 'From');
      | 
      |     for i = 1:length(gotos)
      |         oldTag = get_param(gotos{i}, 'GotoTag');
      |         set_param(gotos{i}, 'GotoTag', regexprep(oldTag, '\d+$', newNum));
      |     end
      |     for i = 1:length(froms)
      |         oldTag = get_param(froms{i}, 'GotoTag');
      |         set_param(froms{i}, 'GotoTag', regexprep(oldTag, '\d+$', newNum));
      |     end
      | 
      |     % --- 2. ПЕРЕИМЕНОВЫВАЕМ САМИ БЛОКИ (визуальные надписи UI0 -> UI1 и т.д.) ---
      |     % Ищем все элементы только внутри этой подсистемы
      |     internalBlocks = find_system(blockPath, 'SearchDepth', 1, 'LookUnderMasks', 'on');
      | 
      |     % Цикл начинаем с 2, так как 1-й элемент в списке - это сама папка подсистемы
      |     for i = 2:length(internalBlocks)
      |         oldName = get_param(internalBlocks{i}, 'Name');
      |         % Ищем цифру в конце имени и меняем на новую
      |         newName = regexprep(oldName, '\d+$', newNum);
      | 
      |         % Если имя изменилось, применяем его
      |         if ~strcmp(oldName, newName)
      |             try
      |                 set_param(internalBlocks{i}, 'Name', newName);
      |             catch
      |                 % Игнорируем ошибку, если вдруг такое имя уже случайно есть
      |             end
      |         end
      |     end
      | end
  M_OUT_Город_6_3 : Subsystem
      settings: CopyFcn=|
      | % Получаем путь и имя нового (только что скопированного) блока
      | blockPath = gcb;
      | blockName = get_param(blockPath, 'Name');
      | 
      | % Ищем число в названии самой подсистемы (например, берем "2" из "Measure_2")
      | numStr = regexp(blockName, '\d+', 'match');
      | 
      | if ~isempty(numStr)
      |     newNum = numStr{end}; % Берем последнее найденное число
      | 
      |     % --- 1. Обновляем скрытые теги в Goto и From (радиочастоты) ---
      |     gotos = find_system(blockPath, 'LookUnderMasks', 'on', 'BlockType', 'Goto');
      |     froms = find_system(blockPath, 'LookUnderMasks', 'on', 'BlockType', 'From');
      | 
      |     for i = 1:length(gotos)
      |         oldTag = get_param(gotos{i}, 'GotoTag');
      |         set_param(gotos{i}, 'GotoTag', regexprep(oldTag, '\d+$', newNum));
      |     end
      |     for i = 1:length(froms)
      |         oldTag = get_param(froms{i}, 'GotoTag');
      |         set_param(froms{i}, 'GotoTag', regexprep(oldTag, '\d+$', newNum));
      |     end
      | 
      |     % --- 2. ПЕРЕИМЕНОВЫВАЕМ САМИ БЛОКИ (визуальные надписи UI0 -> UI1 и т.д.) ---
      |     % Ищем все элементы только внутри этой подсистемы
      |     internalBlocks = find_system(blockPath, 'SearchDepth', 1, 'LookUnderMasks', 'on');
      | 
      |     % Цикл начинаем с 2, так как 1-й элемент в списке - это сама папка подсистемы
      |     for i = 2:length(internalBlocks)
      |         oldName = get_param(internalBlocks{i}, 'Name');
      |         % Ищем цифру в конце имени и меняем на новую
      |         newName = regexprep(oldName, '\d+$', newNum);
      | 
      |         % Если имя изменилось, применяем его
      |         if ~strcmp(oldName, newName)
      |             try
      |                 set_param(internalBlocks{i}, 'Name', newName);
      |             catch
      |                 % Игнорируем ошибку, если вдруг такое имя уже случайно есть
      |             end
      |         end
      |     end
      | end
  M_OUT_Город_6_4 : Subsystem
      settings: CopyFcn=|
      | % Получаем путь и имя нового (только что скопированного) блока
      | blockPath = gcb;
      | blockName = get_param(blockPath, 'Name');
      | 
      | % Ищем число в названии самой подсистемы (например, берем "2" из "Measure_2")
      | numStr = regexp(blockName, '\d+', 'match');
      | 
      | if ~isempty(numStr)
      |     newNum = numStr{end}; % Берем последнее найденное число
      | 
      |     % --- 1. Обновляем скрытые теги в Goto и From (радиочастоты) ---
      |     gotos = find_system(blockPath, 'LookUnderMasks', 'on', 'BlockType', 'Goto');
      |     froms = find_system(blockPath, 'LookUnderMasks', 'on', 'BlockType', 'From');
      | 
      |     for i = 1:length(gotos)
      |         oldTag = get_param(gotos{i}, 'GotoTag');
      |         set_param(gotos{i}, 'GotoTag', regexprep(oldTag, '\d+$', newNum));
      |     end
      |     for i = 1:length(froms)
      |         oldTag = get_param(froms{i}, 'GotoTag');
      |         set_param(froms{i}, 'GotoTag', regexprep(oldTag, '\d+$', newNum));
      |     end
      | 
      |     % --- 2. ПЕРЕИМЕНОВЫВАЕМ САМИ БЛОКИ (визуальные надписи UI0 -> UI1 и т.д.) ---
      |     % Ищем все элементы только внутри этой подсистемы
      |     internalBlocks = find_system(blockPath, 'SearchDepth', 1, 'LookUnderMasks', 'on');
      | 
      |     % Цикл начинаем с 2, так как 1-й элемент в списке - это сама папка подсистемы
      |     for i = 2:length(internalBlocks)
      |         oldName = get_param(internalBlocks{i}, 'Name');
      |         % Ищем цифру в конце имени и меняем на новую
      |         newName = regexprep(oldName, '\d+$', newNum);
      | 
      |         % Если имя изменилось, применяем его
      |         if ~strcmp(oldName, newName)
      |             try
      |                 set_param(internalBlocks{i}, 'Name', newName);
      |             catch
      |                 % Игнорируем ошибку, если вдруг такое имя уже случайно есть
      |             end
      |         end
      |     end
      | end
  M_OUT_Завод_1_1 : Subsystem
      settings: CopyFcn=|
      | % Получаем путь и имя нового (только что скопированного) блока
      | blockPath = gcb;
      | blockName = get_param(blockPath, 'Name');
      | 
      | % Ищем число в названии самой подсистемы (например, берем "2" из "Measure_2")
      | numStr = regexp(blockName, '\d+', 'match');
      | 
      | if ~isempty(numStr)
      |     newNum = numStr{end}; % Берем последнее найденное число
      | 
      |     % --- 1. Обновляем скрытые теги в Goto и From (радиочастоты) ---
      |     gotos = find_system(blockPath, 'LookUnderMasks', 'on', 'BlockType', 'Goto');
      |     froms = find_system(blockPath, 'LookUnderMasks', 'on', 'BlockType', 'From');
      | 
      |     for i = 1:length(gotos)
      |         oldTag = get_param(gotos{i}, 'GotoTag');
      |         set_param(gotos{i}, 'GotoTag', regexprep(oldTag, '\d+$', newNum));
      |     end
      |     for i = 1:length(froms)
      |         oldTag = get_param(froms{i}, 'GotoTag');
      |         set_param(froms{i}, 'GotoTag', regexprep(oldTag, '\d+$', newNum));
      |     end
      | 
      |     % --- 2. ПЕРЕИМЕНОВЫВАЕМ САМИ БЛОКИ (визуальные надписи UI0 -> UI1 и т.д.) ---
      |     % Ищем все элементы только внутри этой подсистемы
      |     internalBlocks = find_system(blockPath, 'SearchDepth', 1, 'LookUnderMasks', 'on');
      | 
      |     % Цикл начинаем с 2, так как 1-й элемент в списке - это сама папка подсистемы
      |     for i = 2:length(internalBlocks)
      |         oldName = get_param(internalBlocks{i}, 'Name');
      |         % Ищем цифру в конце имени и меняем на новую
      |         newName = regexprep(oldName, '\d+$', newNum);
      | 
      |         % Если имя изменилось, применяем его
      |         if ~strcmp(oldName, newName)
      |             try
      |                 set_param(internalBlocks{i}, 'Name', newName);
      |             catch
      |                 % Игнорируем ошибку, если вдруг такое имя уже случайно есть
      |             end
      |         end
      |     end
      | end
  M_OUT_Завод_1_2 : Subsystem
      settings: CopyFcn=|
      | % Получаем путь и имя нового (только что скопированного) блока
      | blockPath = gcb;
      | blockName = get_param(blockPath, 'Name');
      | 
      | % Ищем число в названии самой подсистемы (например, берем "2" из "Measure_2")
      | numStr = regexp(blockName, '\d+', 'match');
      | 
      | if ~isempty(numStr)
      |     newNum = numStr{end}; % Берем последнее найденное число
      | 
      |     % --- 1. Обновляем скрытые теги в Goto и From (радиочастоты) ---
      |     gotos = find_system(blockPath, 'LookUnderMasks', 'on', 'BlockType', 'Goto');
      |     froms = find_system(blockPath, 'LookUnderMasks', 'on', 'BlockType', 'From');
      | 
      |     for i = 1:length(gotos)
      |         oldTag = get_param(gotos{i}, 'GotoTag');
      |         set_param(gotos{i}, 'GotoTag', regexprep(oldTag, '\d+$', newNum));
      |     end
      |     for i = 1:length(froms)
      |         oldTag = get_param(froms{i}, 'GotoTag');
      |         set_param(froms{i}, 'GotoTag', regexprep(oldTag, '\d+$', newNum));
      |     end
      | 
      |     % --- 2. ПЕРЕИМЕНОВЫВАЕМ САМИ БЛОКИ (визуальные надписи UI0 -> UI1 и т.д.) ---
      |     % Ищем все элементы только внутри этой подсистемы
      |     internalBlocks = find_system(blockPath, 'SearchDepth', 1, 'LookUnderMasks', 'on');
      | 
      |     % Цикл начинаем с 2, так как 1-й элемент в списке - это сама папка подсистемы
      |     for i = 2:length(internalBlocks)
      |         oldName = get_param(internalBlocks{i}, 'Name');
      |         % Ищем цифру в конце имени и меняем на новую
      |         newName = regexprep(oldName, '\d+$', newNum);
      | 
      |         % Если имя изменилось, применяем его
      |         if ~strcmp(oldName, newName)
      |             try
      |                 set_param(internalBlocks{i}, 'Name', newName);
      |             catch
      |                 % Игнорируем ошибку, если вдруг такое имя уже случайно есть
      |             end
      |         end
      |     end
      | end
  M_OUT_Завод_2_1 : Subsystem
      settings: CopyFcn=|
      | % Получаем путь и имя нового (только что скопированного) блока
      | blockPath = gcb;
      | blockName = get_param(blockPath, 'Name');
      | 
      | % Ищем число в названии самой подсистемы (например, берем "2" из "Measure_2")
      | numStr = regexp(blockName, '\d+', 'match');
      | 
      | if ~isempty(numStr)
      |     newNum = numStr{end}; % Берем последнее найденное число
      | 
      |     % --- 1. Обновляем скрытые теги в Goto и From (радиочастоты) ---
      |     gotos = find_system(blockPath, 'LookUnderMasks', 'on', 'BlockType', 'Goto');
      |     froms = find_system(blockPath, 'LookUnderMasks', 'on', 'BlockType', 'From');
      | 
      |     for i = 1:length(gotos)
      |         oldTag = get_param(gotos{i}, 'GotoTag');
      |         set_param(gotos{i}, 'GotoTag', regexprep(oldTag, '\d+$', newNum));
      |     end
      |     for i = 1:length(froms)
      |         oldTag = get_param(froms{i}, 'GotoTag');
      |         set_param(froms{i}, 'GotoTag', regexprep(oldTag, '\d+$', newNum));
      |     end
      | 
      |     % --- 2. ПЕРЕИМЕНОВЫВАЕМ САМИ БЛОКИ (визуальные надписи UI0 -> UI1 и т.д.) ---
      |     % Ищем все элементы только внутри этой подсистемы
      |     internalBlocks = find_system(blockPath, 'SearchDepth', 1, 'LookUnderMasks', 'on');
      | 
      |     % Цикл начинаем с 2, так как 1-й элемент в списке - это сама папка подсистемы
      |     for i = 2:length(internalBlocks)
      |         oldName = get_param(internalBlocks{i}, 'Name');
      |         % Ищем цифру в конце имени и меняем на новую
      |         newName = regexprep(oldName, '\d+$', newNum);
      | 
      |         % Если имя изменилось, применяем его
      |         if ~strcmp(oldName, newName)
      |             try
      |                 set_param(internalBlocks{i}, 'Name', newName);
      |             catch
      |                 % Игнорируем ошибку, если вдруг такое имя уже случайно есть
      |             end
      |         end
      |     end
      | end
  M_OUT_Завод_2_2 : Subsystem
      settings: CopyFcn=|
      | % Получаем путь и имя нового (только что скопированного) блока
      | blockPath = gcb;
      | blockName = get_param(blockPath, 'Name');
      | 
      | % Ищем число в названии самой подсистемы (например, берем "2" из "Measure_2")
      | numStr = regexp(blockName, '\d+', 'match');
      | 
      | if ~isempty(numStr)
      |     newNum = numStr{end}; % Берем последнее найденное число
      | 
      |     % --- 1. Обновляем скрытые теги в Goto и From (радиочастоты) ---
      |     gotos = find_system(blockPath, 'LookUnderMasks', 'on', 'BlockType', 'Goto');
      |     froms = find_system(blockPath, 'LookUnderMasks', 'on', 'BlockType', 'From');
      | 
      |     for i = 1:length(gotos)
      |         oldTag = get_param(gotos{i}, 'GotoTag');
      |         set_param(gotos{i}, 'GotoTag', regexprep(oldTag, '\d+$', newNum));
      |     end
      |     for i = 1:length(froms)
      |         oldTag = get_param(froms{i}, 'GotoTag');
      |         set_param(froms{i}, 'GotoTag', regexprep(oldTag, '\d+$', newNum));
      |     end
      | 
      |     % --- 2. ПЕРЕИМЕНОВЫВАЕМ САМИ БЛОКИ (визуальные надписи UI0 -> UI1 и т.д.) ---
      |     % Ищем все элементы только внутри этой подсистемы
      |     internalBlocks = find_system(blockPath, 'SearchDepth', 1, 'LookUnderMasks', 'on');
      | 
      |     % Цикл начинаем с 2, так как 1-й элемент в списке - это сама папка подсистемы
      |     for i = 2:length(internalBlocks)
      |         oldName = get_param(internalBlocks{i}, 'Name');
      |         % Ищем цифру в конце имени и меняем на новую
      |         newName = regexprep(oldName, '\d+$', newNum);
      | 
      |         % Если имя изменилось, применяем его
      |         if ~strcmp(oldName, newName)
      |             try
      |                 set_param(internalBlocks{i}, 'Name', newName);
      |             catch
      |                 % Игнорируем ошибку, если вдруг такое имя уже случайно есть
      |             end
      |         end
      |     end
      | end
  M_OUT_Завод_3_1 : Subsystem
      settings: CopyFcn=|
      | % Получаем путь и имя нового (только что скопированного) блока
      | blockPath = gcb;
      | blockName = get_param(blockPath, 'Name');
      | 
      | % Ищем число в названии самой подсистемы (например, берем "2" из "Measure_2")
      | numStr = regexp(blockName, '\d+', 'match');
      | 
      | if ~isempty(numStr)
      |     newNum = numStr{end}; % Берем последнее найденное число
      | 
      |     % --- 1. Обновляем скрытые теги в Goto и From (радиочастоты) ---
      |     gotos = find_system(blockPath, 'LookUnderMasks', 'on', 'BlockType', 'Goto');
      |     froms = find_system(blockPath, 'LookUnderMasks', 'on', 'BlockType', 'From');
      | 
      |     for i = 1:length(gotos)
      |         oldTag = get_param(gotos{i}, 'GotoTag');
      |         set_param(gotos{i}, 'GotoTag', regexprep(oldTag, '\d+$', newNum));
      |     end
      |     for i = 1:length(froms)
      |         oldTag = get_param(froms{i}, 'GotoTag');
      |         set_param(froms{i}, 'GotoTag', regexprep(oldTag, '\d+$', newNum));
      |     end
      | 
      |     % --- 2. ПЕРЕИМЕНОВЫВАЕМ САМИ БЛОКИ (визуальные надписи UI0 -> UI1 и т.д.) ---
      |     % Ищем все элементы только внутри этой подсистемы
      |     internalBlocks = find_system(blockPath, 'SearchDepth', 1, 'LookUnderMasks', 'on');
      | 
      |     % Цикл начинаем с 2, так как 1-й элемент в списке - это сама папка подсистемы
      |     for i = 2:length(internalBlocks)
      |         oldName = get_param(internalBlocks{i}, 'Name');
      |         % Ищем цифру в конце имени и меняем на новую
      |         newName = regexprep(oldName, '\d+$', newNum);
      | 
      |         % Если имя изменилось, применяем его
      |         if ~strcmp(oldName, newName)
      |             try
      |                 set_param(internalBlocks{i}, 'Name', newName);
      |             catch
      |                 % Игнорируем ошибку, если вдруг такое имя уже случайно есть
      |             end
      |         end
      |     end
      | end
  M_OUT_Завод_3_2 : Subsystem
      settings: CopyFcn=|
      | % Получаем путь и имя нового (только что скопированного) блока
      | blockPath = gcb;
      | blockName = get_param(blockPath, 'Name');
      | 
      | % Ищем число в названии самой подсистемы (например, берем "2" из "Measure_2")
      | numStr = regexp(blockName, '\d+', 'match');
      | 
      | if ~isempty(numStr)
      |     newNum = numStr{end}; % Берем последнее найденное число
      | 
      |     % --- 1. Обновляем скрытые теги в Goto и From (радиочастоты) ---
      |     gotos = find_system(blockPath, 'LookUnderMasks', 'on', 'BlockType', 'Goto');
      |     froms = find_system(blockPath, 'LookUnderMasks', 'on', 'BlockType', 'From');
      | 
      |     for i = 1:length(gotos)
      |         oldTag = get_param(gotos{i}, 'GotoTag');
      |         set_param(gotos{i}, 'GotoTag', regexprep(oldTag, '\d+$', newNum));
      |     end
      |     for i = 1:length(froms)
      |         oldTag = get_param(froms{i}, 'GotoTag');
      |         set_param(froms{i}, 'GotoTag', regexprep(oldTag, '\d+$', newNum));
      |     end
      | 
      |     % --- 2. ПЕРЕИМЕНОВЫВАЕМ САМИ БЛОКИ (визуальные надписи UI0 -> UI1 и т.д.) ---
      |     % Ищем все элементы только внутри этой подсистемы
      |     internalBlocks = find_system(blockPath, 'SearchDepth', 1, 'LookUnderMasks', 'on');
      | 
      |     % Цикл начинаем с 2, так как 1-й элемент в списке - это сама папка подсистемы
      |     for i = 2:length(internalBlocks)
      |         oldName = get_param(internalBlocks{i}, 'Name');
      |         % Ищем цифру в конце имени и меняем на новую
      |         newName = regexprep(oldName, '\d+$', newNum);
      | 
      |         % Если имя изменилось, применяем его
      |         if ~strcmp(oldName, newName)
      |             try
      |                 set_param(internalBlocks{i}, 'Name', newName);
      |             catch
      |                 % Игнорируем ошибку, если вдруг такое имя уже случайно есть
      |             end
      |         end
      |     end
      | end
  M_OUT_Завод_4_1 : Subsystem
      settings: CopyFcn=|
      | % Получаем путь и имя нового (только что скопированного) блока
      | blockPath = gcb;
      | blockName = get_param(blockPath, 'Name');
      | 
      | % Ищем число в названии самой подсистемы (например, берем "2" из "Measure_2")
      | numStr = regexp(blockName, '\d+', 'match');
      | 
      | if ~isempty(numStr)
      |     newNum = numStr{end}; % Берем последнее найденное число
      | 
      |     % --- 1. Обновляем скрытые теги в Goto и From (радиочастоты) ---
      |     gotos = find_system(blockPath, 'LookUnderMasks', 'on', 'BlockType', 'Goto');
      |     froms = find_system(blockPath, 'LookUnderMasks', 'on', 'BlockType', 'From');
      | 
      |     for i = 1:length(gotos)
      |         oldTag = get_param(gotos{i}, 'GotoTag');
      |         set_param(gotos{i}, 'GotoTag', regexprep(oldTag, '\d+$', newNum));
      |     end
      |     for i = 1:length(froms)
      |         oldTag = get_param(froms{i}, 'GotoTag');
      |         set_param(froms{i}, 'GotoTag', regexprep(oldTag, '\d+$', newNum));
      |     end
      | 
      |     % --- 2. ПЕРЕИМЕНОВЫВАЕМ САМИ БЛОКИ (визуальные надписи UI0 -> UI1 и т.д.) ---
      |     % Ищем все элементы только внутри этой подсистемы
      |     internalBlocks = find_system(blockPath, 'SearchDepth', 1, 'LookUnderMasks', 'on');
      | 
